simulink model "model"  (R2014a)
(part 6 of 6)

  _CN_132159930_220000_CN_132517028_220000/RConn3 -- T_132517028__Ruwais/LConn3 -- _CN_95139157_220000_CN_132517028_220000/LConn3 -- bus236/LConn1
  _CN_247122500_220000_CN_354672632_220000/LConn1 -- T_247122500__/LConn1 -- _CN_247122500_220000_CN_115677414_220000/LConn1
  _CN_247122500_220000_CN_354672632_220000/LConn2 -- T_247122500__/LConn2 -- _CN_247122500_220000_CN_115677414_220000/LConn2
  _CN_247122500_220000_CN_354672632_220000/LConn3 -- T_247122500__/LConn3 -- _CN_247122500_220000_CN_115677414_220000/LConn3 -- bus237/LConn1
  _CN_247122500_220000_CN_354672632_220000/RConn1 -- T_354672632__/LConn1 -- _CN_60234385_220000_CN_354672632_220000/LConn1 -- _CN_115677414_220000_CN_354672632_220000/LConn1
  _CN_247122500_220000_CN_354672632_220000/RConn2 -- T_354672632__/LConn2 -- _CN_60234385_220000_CN_354672632_220000/LConn2 -- _CN_115677414_220000_CN_354672632_220000/LConn2
  _CN_247122500_220000_CN_354672632_220000/RConn3 -- T_354672632__/LConn3 -- _CN_60234385_220000_CN_354672632_220000/LConn3 -- bus238/LConn1 -- _CN_115677414_220000_CN_354672632_220000/LConn3
  _CN_247122500_220000_CN_115677414_220000/RConn1 -- T_115677414__/LConn1 -- _CN_354672631_220000_CN_115677414_220000/RConn1 -- _CN_115677398_220000_CN_115677414_220000/LConn1 -- _CN_115677414_220000_CN_386199541_220000/LConn1 -- _CN_115677414_220000_CN_354672632_220000/RConn1
  _CN_247122500_220000_CN_115677414_220000/RConn2 -- T_115677414__/LConn2 -- _CN_354672631_220000_CN_115677414_220000/RConn2 -- _CN_115677398_220000_CN_115677414_220000/LConn2 -- _CN_115677414_220000_CN_386199541_220000/LConn2 -- _CN_115677414_220000_CN_354672632_220000/RConn2
  _CN_247122500_220000_CN_115677414_220000/RConn3 -- T_115677414__/LConn3 -- _CN_354672631_220000_CN_115677414_220000/RConn3 -- _CN_115677398_220000_CN_115677414_220000/LConn3 -- _CN_115677414_220000_CN_386199541_220000/LConn3 -- _CN_115677414_220000_CN_354672632_220000/RConn3 -- bus239/LConn1
  T_95099973__Liwa/LConn1 -- _CN_95099973_220000_CN_95099964_220000/RConn1
  T_95099973__Liwa/LConn2 -- _CN_95099973_220000_CN_95099964_220000/RConn2
  _CN_95099973_220000_CN_95099964_220000/RConn3 -- T_95099973__Liwa/LConn3 -- bus240/LConn1
  _CN_95139157_220000_CN_132517028_220000/RConn1 -- T_95139157__Shuweihat/RConn1 -- L_95139157/LConn1
  _CN_95139157_220000_CN_132517028_220000/RConn2 -- T_95139157__Shuweihat/RConn2 -- L_95139157/LConn2
  _CN_95139157_220000_CN_132517028_220000/RConn3 -- T_95139157__Shuweihat/RConn3 -- L_95139157/LConn3 -- bus241/LConn1
  _CN_115677398_220000_CN_115677409_220000/LConn1 -- T_115677398__/LConn1 -- _CN_115677398_220000_CN_386199534_220000/LConn1 -- _CN_115677398_220000_CN_115677414_220000/RConn1 -- _CN_115677398_220000_CN_386199505_220000/LConn1
  _CN_115677398_220000_CN_115677409_220000/LConn2 -- T_115677398__/LConn2 -- _CN_115677398_220000_CN_386199534_220000/LConn2 -- _CN_115677398_220000_CN_115677414_220000/RConn2 -- _CN_115677398_220000_CN_386199505_220000/LConn2
  _CN_115677398_220000_CN_115677409_220000/LConn3 -- T_115677398__/LConn3 -- _CN_115677398_220000_CN_386199534_220000/LConn3 -- _CN_115677398_220000_CN_115677414_220000/RConn3 -- bus242/LConn1 -- _CN_115677398_220000_CN_386199505_220000/LConn3
  G_115677409_/RConn1 -- _CN_115677398_220000_CN_115677409_220000/RConn1
  G_115677409_/RConn2 -- _CN_115677398_220000_CN_115677409_220000/RConn2
  _CN_115677398_220000_CN_115677409_220000/RConn3 -- G_115677409_/RConn3 -- bus243/LConn1
  G_386199505_/RConn1 -- _CN_115677398_220000_CN_386199505_220000/RConn1
  G_386199505_/RConn2 -- _CN_115677398_220000_CN_386199505_220000/RConn2
  _CN_115677398_220000_CN_386199505_220000/RConn3 -- G_386199505_/RConn3 -- bus244/LConn1
  _CN_115677398_220000_CN_386199534_220000/RConn1 -- T_386199534__/LConn1 -- _CN_386199534_220000_CN_386199541_220000/LConn1
  _CN_115677398_220000_CN_386199534_220000/RConn2 -- T_386199534__/LConn2 -- _CN_386199534_220000_CN_386199541_220000/LConn2
  _CN_115677398_220000_CN_386199534_220000/RConn3 -- T_386199534__/LConn3 -- _CN_386199534_220000_CN_386199541_220000/LConn3 -- bus245/LConn1
  _CN_200057688_220000_CN_95084793_220000/RConn1 -- T_95084793__/LConn1 -- _CN_95084771_220000_CN_95084793_220000/RConn1
  _CN_200057688_220000_CN_95084793_220000/RConn2 -- T_95084793__/LConn2 -- _CN_95084771_220000_CN_95084793_220000/RConn2
  _CN_200057688_220000_CN_95084793_220000/RConn3 -- T_95084793__/LConn3 -- _CN_95084771_220000_CN_95084793_220000/RConn3 -- bus246/LConn1
  _CN_115677414_220000_CN_386199541_220000/RConn1 -- T_386199541__/LConn1 -- _CN_386199534_220000_CN_386199541_220000/RConn1
  _CN_115677414_220000_CN_386199541_220000/RConn2 -- T_386199541__/LConn2 -- _CN_386199534_220000_CN_386199541_220000/RConn2
  _CN_115677414_220000_CN_386199541_220000/RConn3 -- T_386199541__/LConn3 -- _CN_386199534_220000_CN_386199541_220000/RConn3 -- bus247/LConn1
  T_60234385__/LConn1 -- _CN_60234385_220000_CN_354672632_220000/RConn1
  T_60234385__/LConn2 -- _CN_60234385_220000_CN_354672632_220000/RConn2
  _CN_60234385_220000_CN_354672632_220000/RConn3 -- T_60234385__/LConn3 -- bus248/LConn1
  _CN_95099964_220000_CN_95139199_220000/RConn1 -- T_95139199__Mirfa/RConn1 -- L_95139199/LConn1
  _CN_95099964_220000_CN_95139199_220000/RConn2 -- T_95139199__Mirfa/RConn2 -- L_95139199/LConn2
  _CN_95099964_220000_CN_95139199_220000/RConn3 -- T_95139199__Mirfa/RConn3 -- L_95139199/LConn3 -- bus249/LConn1
  T_198365955__/LConn1 -- _CN_198365955_230000_CN_199091189_230000/LConn1
  T_198365955__/LConn2 -- _CN_198365955_230000_CN_199091189_230000/LConn2
  _CN_198365955_230000_CN_199091189_230000/LConn3 -- T_198365955__/LConn3 -- bus250/LConn1
  T_199091189__/LConn1 -- _CN_198365955_230000_CN_199091189_230000/RConn1
  T_199091189__/LConn2 -- _CN_198365955_230000_CN_199091189_230000/RConn2
  _CN_198365955_230000_CN_199091189_230000/RConn3 -- T_199091189__/LConn3 -- bus251/LConn1
  T_46971910__/LConn1 -- _CN_46971910_230000_CN_197436611_230000/LConn1
  T_46971910__/LConn2 -- _CN_46971910_230000_CN_197436611_230000/LConn2
  _CN_46971910_230000_CN_197436611_230000/LConn3 -- T_46971910__/LConn3 -- bus252/LConn1
  _CN_46971910_230000_CN_197436611_230000/RConn1 -- G_197436611_/RConn1 -- _CN_197445313_230000_CN_197436611_230000/LConn1 -- _CN_132976488_230000_CN_197436611_230000/LConn1 -- _CN_197662314_230000_CN_197436611_230000/LConn1 -- _CN_197432428_230000_CN_197436611_230000/LConn1 -- _CN_132978605_380000_CN_197436611_230000/LConn1 -- _CN_197252542_380000_CN_197436611_230000/LConn1
  _CN_46971910_230000_CN_197436611_230000/RConn2 -- G_197436611_/RConn2 -- _CN_197445313_230000_CN_197436611_230000/LConn2 -- _CN_132976488_230000_CN_197436611_230000/LConn2 -- _CN_197662314_230000_CN_197436611_230000/LConn2 -- _CN_197432428_230000_CN_197436611_230000/LConn2 -- _CN_132978605_380000_CN_197436611_230000/LConn2 -- _CN_197252542_380000_CN_197436611_230000/LConn2
  _CN_46971910_230000_CN_197436611_230000/RConn3 -- G_197436611_/RConn3 -- _CN_197445313_230000_CN_197436611_230000/LConn3 -- _CN_132976488_230000_CN_197436611_230000/LConn3 -- _CN_197662314_230000_CN_197436611_230000/LConn3 -- _CN_197432428_230000_CN_197436611_230000/LConn3 -- _CN_132978605_380000_CN_197436611_230000/LConn3 -- _CN_197252542_380000_CN_197436611_230000/LConn3 -- bus253/LConn1
  _CN_198351119_230000_CN_198331310_230000/LConn1 -- T_198351119__/LConn1 -- _CN_198351119_230000_CN_198330048_230000/LConn1 -- _CN_198351119_230000_CN_132978605_230000/LConn1 -- _CN_198351119_230000_CN_132976488_230000/LConn1 -- _CN_198351119_230000_CN_198342216_230000/LConn1
  _CN_198351119_230000_CN_198331310_230000/LConn2 -- T_198351119__/LConn2 -- _CN_198351119_230000_CN_198330048_230000/LConn2 -- _CN_198351119_230000_CN_132978605_230000/LConn2 -- _CN_198351119_230000_CN_132976488_230000/LConn2 -- _CN_198351119_230000_CN_198342216_230000/LConn2
  _CN_198351119_230000_CN_198331310_230000/LConn3 -- T_198351119__/LConn3 -- _CN_198351119_230000_CN_198330048_230000/LConn3 -- _CN_198351119_230000_CN_132978605_230000/LConn3 -- _CN_198351119_230000_CN_132976488_230000/LConn3 -- _CN_198351119_230000_CN_198342216_230000/LConn3 -- bus254/LConn1
  _CN_198351119_230000_CN_198331310_230000/RConn1 -- T_198331310__/LConn1 -- _CN_198334634_230000_CN_198331310_230000/LConn1 -- _CN_132978605_230000_CN_198331310_230000/LConn1
  _CN_198351119_230000_CN_198331310_230000/RConn2 -- T_198331310__/LConn2 -- _CN_198334634_230000_CN_198331310_230000/LConn2 -- _CN_132978605_230000_CN_198331310_230000/LConn2
  _CN_198351119_230000_CN_198331310_230000/RConn3 -- T_198331310__/LConn3 -- _CN_198334634_230000_CN_198331310_230000/LConn3 -- _CN_132978605_230000_CN_198331310_230000/LConn3 -- bus255/LConn1
  T_198330048__/LConn1 -- _CN_198351119_230000_CN_198330048_230000/RConn1
  T_198330048__/LConn2 -- _CN_198351119_230000_CN_198330048_230000/RConn2
  _CN_198351119_230000_CN_198330048_230000/RConn3 -- T_198330048__/LConn3 -- bus256/LConn1
  _CN_198351119_230000_CN_132978605_230000/RConn1 -- T_132978605__/RConn1 -- _CN_132978605_230000_CN_198144511_230000/LConn1 -- _CN_132978605_230000_CN_198331310_230000/RConn1 -- L_132978605/LConn1
  _CN_198351119_230000_CN_132978605_230000/RConn2 -- T_132978605__/RConn2 -- _CN_132978605_230000_CN_198144511_230000/LConn2 -- _CN_132978605_230000_CN_198331310_230000/RConn2 -- L_132978605/LConn2
  _CN_198351119_230000_CN_132978605_230000/RConn3 -- T_132978605__/RConn3 -- _CN_132978605_230000_CN_198144511_230000/LConn3 -- _CN_132978605_230000_CN_198331310_230000/RConn3 -- L_132978605/LConn3 -- bus257/LConn1
  _CN_198351119_230000_CN_132976488_230000/RConn1 -- T_132976488__Berri_Gas_Plant/LConn1 -- _CN_132976488_230000_CN_197436611_230000/RConn1 -- _CN_132976488_230000_CN_198144511_230000/LConn1
  _CN_198351119_230000_CN_132976488_230000/RConn2 -- T_132976488__Berri_Gas_Plant/LConn2 -- _CN_132976488_230000_CN_197436611_230000/RConn2 -- _CN_132976488_230000_CN_198144511_230000/LConn2
  _CN_198351119_230000_CN_132976488_230000/RConn3 -- T_132976488__Berri_Gas_Plant/LConn3 -- _CN_132976488_230000_CN_197436611_230000/RConn3 -- bus258/LConn1 -- _CN_132976488_230000_CN_198144511_230000/LConn3
  T_198342216__/LConn1 -- _CN_198351119_230000_CN_198342216_230000/RConn1
  T_198342216__/LConn2 -- _CN_198351119_230000_CN_198342216_230000/RConn2
  _CN_198351119_230000_CN_198342216_230000/RConn3 -- T_198342216__/LConn3 -- bus259/LConn1
  _CN_168652821_230000_CN_198358326_230000/LConn1 -- T_168652821__/LConn1 -- _CN_168652821_230000_CN_188546296_230000/LConn1
  _CN_168652821_230000_CN_198358326_230000/LConn2 -- T_168652821__/LConn2 -- _CN_168652821_230000_CN_188546296_230000/LConn2
  _CN_168652821_230000_CN_198358326_230000/LConn3 -- T_168652821__/LConn3 -- _CN_168652821_230000_CN_188546296_230000/LConn3 -- bus260/LConn1
  T_198358326__/LConn1 -- _CN_168652821_230000_CN_198358326_230000/RConn1
  T_198358326__/LConn2 -- _CN_168652821_230000_CN_198358326_230000/RConn2
  _CN_168652821_230000_CN_198358326_230000/RConn3 -- T_198358326__/LConn3 -- bus261/LConn1
  T_188546296__/LConn1 -- _CN_168652821_230000_CN_188546296_230000/RConn1
  T_188546296__/LConn2 -- _CN_168652821_230000_CN_188546296_230000/RConn2
  _CN_168652821_230000_CN_188546296_230000/RConn3 -- T_188546296__/LConn3 -- bus262/LConn1
  T_198334634__/LConn1 -- _CN_198334634_230000_CN_198331310_230000/RConn1
  T_198334634__/LConn2 -- _CN_198334634_230000_CN_198331310_230000/RConn2
  _CN_198334634_230000_CN_198331310_230000/RConn3 -- T_198334634__/LConn3 -- bus263/LConn1
  _CN_132978605_230000_CN_198144511_230000/RConn1 -- T_198144511__/LConn1 -- _CN_197662314_230000_CN_198144511_230000/LConn1 -- _CN_132976488_230000_CN_198144511_230000/RConn1
  _CN_132978605_230000_CN_198144511_230000/RConn2 -- T_198144511__/LConn2 -- _CN_197662314_230000_CN_198144511_230000/LConn2 -- _CN_132976488_230000_CN_198144511_230000/RConn2
  _CN_132978605_230000_CN_198144511_230000/RConn3 -- T_198144511__/LConn3 -- _CN_197662314_230000_CN_198144511_230000/LConn3 -- bus264/LConn1 -- _CN_132976488_230000_CN_198144511_230000/RConn3
  T_195637944__/LConn1 -- _CN_195637944_230000_CN_115326815_230000/LConn1
  T_195637944__/LConn2 -- _CN_195637944_230000_CN_115326815_230000/LConn2
  _CN_195637944_230000_CN_115326815_230000/LConn3 -- T_195637944__/LConn3 -- bus265/LConn1
  _CN_195637944_230000_CN_115326815_230000/RConn1 -- T_115326815_380000_/RConn1 -- _CN_115326815_230000_CN_115326819_230000/LConn1 -- L_115326815/LConn1 -- _CN_168648926_230000_CN_115326815_230000/LConn1
  _CN_195637944_230000_CN_115326815_230000/RConn2 -- T_115326815_380000_/RConn2 -- _CN_115326815_230000_CN_115326819_230000/LConn2 -- L_115326815/LConn2 -- _CN_168648926_230000_CN_115326815_230000/LConn2
  _CN_195637944_230000_CN_115326815_230000/RConn3 -- T_115326815_380000_/RConn3 -- _CN_115326815_230000_CN_115326819_230000/LConn3 -- L_115326815/LConn3 -- bus266/LConn1 -- _CN_168648926_230000_CN_115326815_230000/LConn3
  T_197445313__/LConn1 -- _CN_197445313_230000_CN_197436611_230000/RConn1
  T_197445313__/LConn2 -- _CN_197445313_230000_CN_197436611_230000/RConn2
  _CN_197445313_230000_CN_197436611_230000/RConn3 -- T_197445313__/LConn3 -- bus267/LConn1
  T_168648926__/LConn1 -- _CN_168648926_230000_CN_115326815_230000/RConn1
  T_168648926__/LConn2 -- _CN_168648926_230000_CN_115326815_230000/RConn2
  _CN_168648926_230000_CN_115326815_230000/RConn3 -- T_168648926__/LConn3 -- bus268/LConn1
  T_115326819__/LConn1 -- _CN_115326815_230000_CN_115326819_230000/RConn1
  T_115326819__/LConn2 -- _CN_115326815_230000_CN_115326819_230000/RConn2
  _CN_115326815_230000_CN_115326819_230000/RConn3 -- T_115326819__/LConn3 -- bus269/LConn1
  _CN_197662314_230000_CN_198144511_230000/RConn1 -- T_197662314__/LConn1 -- _CN_197662314_230000_CN_197436611_230000/RConn1
  _CN_197662314_230000_CN_198144511_230000/RConn2 -- T_197662314__/LConn2 -- _CN_197662314_230000_CN_197436611_230000/RConn2
  _CN_197662314_230000_CN_198144511_230000/RConn3 -- T_197662314__/LConn3 -- _CN_197662314_230000_CN_197436611_230000/RConn3 -- bus270/LConn1
  _CN_197432428_230000_CN_197442799_230000/LConn1 -- T_197432428__/LConn1 -- _CN_197432428_230000_CN_197439486_230000/LConn1 -- _CN_197432428_230000_CN_197436611_230000/RConn1
  _CN_197432428_230000_CN_197442799_230000/LConn2 -- T_197432428__/LConn2 -- _CN_197432428_230000_CN_197439486_230000/LConn2 -- _CN_197432428_230000_CN_197436611_230000/RConn2
  _CN_197432428_230000_CN_197442799_230000/LConn3 -- T_197432428__/LConn3 -- _CN_197432428_230000_CN_197439486_230000/LConn3 -- bus271/LConn1 -- _CN_197432428_230000_CN_197436611_230000/RConn3
  T_197442799__/LConn1 -- _CN_197432428_230000_CN_197442799_230000/RConn1
  T_197442799__/LConn2 -- _CN_197432428_230000_CN_197442799_230000/RConn2
  _CN_197432428_230000_CN_197442799_230000/RConn3 -- T_197442799__/LConn3 -- bus272/LConn1
  T_197439486__/LConn1 -- _CN_197432428_230000_CN_197439486_230000/RConn1
  T_197439486__/LConn2 -- _CN_197432428_230000_CN_197439486_230000/RConn2
  _CN_197432428_230000_CN_197439486_230000/RConn3 -- T_197439486__/LConn3 -- bus273/LConn1
  T_261938325__/LConn1 -- _CN_261938325_275000_CN_160398714_275000/LConn1
  T_261938325__/LConn2 -- _CN_261938325_275000_CN_160398714_275000/LConn2
  _CN_261938325_275000_CN_160398714_275000/LConn3 -- T_261938325__/LConn3 -- bus274/LConn1
  _CN_261938325_275000_CN_160398714_275000/RConn1 -- T_160398714__/LConn1 -- _CN_261938316_275000_CN_160398714_275000/LConn1
  _CN_261938325_275000_CN_160398714_275000/RConn2 -- T_160398714__/LConn2 -- _CN_261938316_275000_CN_160398714_275000/LConn2
  _CN_261938325_275000_CN_160398714_275000/RConn3 -- T_160398714__/LConn3 -- _CN_261938316_275000_CN_160398714_275000/LConn3 -- bus275/LConn1
  T_203618603__/LConn1 -- _CN_203618603_275000_CN_132154027_275000/LConn1
  T_203618603__/LConn2 -- _CN_203618603_275000_CN_132154027_275000/LConn2
  _CN_203618603_275000_CN_132154027_275000/LConn3 -- T_203618603__/LConn3 -- bus276/LConn1
  _CN_203618603_275000_CN_132154027_275000/RConn1 -- T_132154027__/LConn1 -- _CN_203622086_275000_CN_132154027_275000/LConn1 -- _CN_132154027_275000_CN_204277162_275000/LConn1 -- _CN_132154027_275000_CN_203855651_275000/LConn1 -- _CN_132154027_275000_CN_132889809_275000/LConn1 -- _CN_132154027_275000_CN_132154028_275000/LConn1
  _CN_203618603_275000_CN_132154027_275000/RConn2 -- T_132154027__/LConn2 -- _CN_203622086_275000_CN_132154027_275000/LConn2 -- _CN_132154027_275000_CN_204277162_275000/LConn2 -- _CN_132154027_275000_CN_203855651_275000/LConn2 -- _CN_132154027_275000_CN_132889809_275000/LConn2 -- _CN_132154027_275000_CN_132154028_275000/LConn2
  _CN_203618603_275000_CN_132154027_275000/RConn3 -- T_132154027__/LConn3 -- _CN_203622086_275000_CN_132154027_275000/LConn3 -- _CN_132154027_275000_CN_204277162_275000/LConn3 -- _CN_132154027_275000_CN_203855651_275000/LConn3 -- _CN_132154027_275000_CN_132889809_275000/LConn3 -- _CN_132154027_275000_CN_132154028_275000/LConn3 -- bus277/LConn1
  T_203622084__/LConn1 -- _CN_203622084_275000_CN_204277162_275000/LConn1
  T_203622084__/LConn2 -- _CN_203622084_275000_CN_204277162_275000/LConn2
  _CN_203622084_275000_CN_204277162_275000/LConn3 -- T_203622084__/LConn3 -- bus278/LConn1
  _CN_203622084_275000_CN_204277162_275000/RConn1 -- G_204277162_Al_Zour_Thermal_Power_Plant/RConn1 -- _CN_132154027_275000_CN_204277162_275000/RConn1 -- _CN_204276494_275000_CN_204277162_275000/LConn1 -- _CN_203618746_275000_CN_204277162_275000/LConn1
  _CN_203622084_275000_CN_204277162_275000/RConn2 -- G_204277162_Al_Zour_Thermal_Power_Plant/RConn2 -- _CN_132154027_275000_CN_204277162_275000/RConn2 -- _CN_204276494_275000_CN_204277162_275000/LConn2 -- _CN_203618746_275000_CN_204277162_275000/LConn2
  _CN_203622084_275000_CN_204277162_275000/RConn3 -- G_204277162_Al_Zour_Thermal_Power_Plant/RConn3 -- _CN_132154027_275000_CN_204277162_275000/RConn3 -- _CN_204276494_275000_CN_204277162_275000/LConn3 -- _CN_203618746_275000_CN_204277162_275000/LConn3 -- bus279/LConn1
  T_203622086__/LConn1 -- _CN_203622086_275000_CN_132154027_275000/RConn1
  T_203622086__/LConn2 -- _CN_203622086_275000_CN_132154027_275000/RConn2
  _CN_203622086_275000_CN_132154027_275000/RConn3 -- T_203622086__/LConn3 -- bus280/LConn1
  T_203622279__/LConn1 -- _CN_203622279_275000_CN_132889809_275000/LConn1
  T_203622279__/LConn2 -- _CN_203622279_275000_CN_132889809_275000/LConn2
  _CN_203622279_275000_CN_132889809_275000/LConn3 -- T_203622279__/LConn3 -- bus281/LConn1
  _CN_203622279_275000_CN_132889809_275000/RConn1 -- T_132889809__/LConn1 -- _CN_132154027_275000_CN_132889809_275000/RConn1 -- _CN_203858094_275000_CN_132889809_275000/LConn1
  _CN_203622279_275000_CN_132889809_275000/RConn2 -- T_132889809__/LConn2 -- _CN_132154027_275000_CN_132889809_275000/RConn2 -- _CN_203858094_275000_CN_132889809_275000/LConn2
  _CN_203622279_275000_CN_132889809_275000/RConn3 -- T_132889809__/LConn3 -- _CN_132154027_275000_CN_132889809_275000/RConn3 -- _CN_203858094_275000_CN_132889809_275000/LConn3 -- bus282/LConn1
  "T_261938316__Substation_Al_Omariya_\"W\""/LConn1 -- _CN_261938316_275000_CN_160398714_275000/RConn1
  "T_261938316__Substation_Al_Omariya_\"W\""/LConn2 -- _CN_261938316_275000_CN_160398714_275000/RConn2
  _CN_261938316_275000_CN_160398714_275000/RConn3 -- "T_261938316__Substation_Al_Omariya_\"W\""/LConn3 -- bus283/LConn1
  _CN_132154027_275000_CN_203855651_275000/RConn1 -- T_203855651__/LConn1 -- _CN_132154028_275000_CN_203855651_275000/LConn1
  _CN_132154027_275000_CN_203855651_275000/RConn2 -- T_203855651__/LConn2 -- _CN_132154028_275000_CN_203855651_275000/LConn2
  _CN_132154027_275000_CN_203855651_275000/RConn3 -- T_203855651__/LConn3 -- _CN_132154028_275000_CN_203855651_275000/LConn3 -- bus284/LConn1
  _CN_132154027_275000_CN_132154028_275000/RConn1 -- T_132154028__Substation/LConn1 -- _CN_132154028_275000_CN_203855651_275000/RConn1
  _CN_132154027_275000_CN_132154028_275000/RConn2 -- T_132154028__Substation/LConn2 -- _CN_132154028_275000_CN_203855651_275000/RConn2
  _CN_132154027_275000_CN_132154028_275000/RConn3 -- T_132154028__Substation/LConn3 -- _CN_132154028_275000_CN_203855651_275000/RConn3 -- bus285/LConn1
  T_203858094__/LConn1 -- _CN_203858094_275000_CN_132889809_275000/RConn1
  T_203858094__/LConn2 -- _CN_203858094_275000_CN_132889809_275000/RConn2
  _CN_203858094_275000_CN_132889809_275000/RConn3 -- T_203858094__/LConn3 -- bus286/LConn1
  _CN_204276494_275000_CN_204277162_275000/RConn1 -- T_204276494__/RConn1 -- L_204276494/LConn1
  _CN_204276494_275000_CN_204277162_275000/RConn2 -- T_204276494__/RConn2 -- L_204276494/LConn2
  _CN_204276494_275000_CN_204277162_275000/RConn3 -- T_204276494__/RConn3 -- L_204276494/LConn3 -- bus287/LConn1
  T_203618746__/LConn1 -- _CN_203618746_275000_CN_204277162_275000/RConn1
  T_203618746__/LConn2 -- _CN_203618746_275000_CN_204277162_275000/RConn2
  _CN_203618746_275000_CN_204277162_275000/RConn3 -- T_203618746__/LConn3 -- bus288/LConn1
  _CN_196903043_380000_CN_115345577_380000/LConn1 -- T_196903043__/LConn1 -- _CN_196903043_380000_CN_115326815_380000/LConn1 -- _CN_196903043_380000_CN_196917881_380000/LConn1
  _CN_196903043_380000_CN_115345577_380000/LConn2 -- T_196903043__/LConn2 -- _CN_196903043_380000_CN_115326815_380000/LConn2 -- _CN_196903043_380000_CN_196917881_380000/LConn2
  _CN_196903043_380000_CN_115345577_380000/LConn3 -- T_196903043__/LConn3 -- _CN_196903043_380000_CN_115326815_380000/LConn3 -- _CN_196903043_380000_CN_196917881_380000/LConn3 -- bus289/LConn1
  _CN_196903043_380000_CN_115345577_380000/RConn1 -- T_115345577__/LConn1 -- _CN_115345577_380000_CN_195636040_380000/LConn1 -- _CN_115345577_380000_CN_115326815_380000/LConn1
  _CN_196903043_380000_CN_115345577_380000/RConn2 -- T_115345577__/LConn2 -- _CN_115345577_380000_CN_195636040_380000/LConn2 -- _CN_115345577_380000_CN_115326815_380000/LConn2
  _CN_196903043_380000_CN_115345577_380000/RConn3 -- T_115345577__/LConn3 -- _CN_115345577_380000_CN_195636040_380000/LConn3 -- _CN_115345577_380000_CN_115326815_380000/LConn3 -- bus290/LConn1
  _CN_196903043_380000_CN_115326815_380000/RConn1 -- T_115326815_380000_/LConn1 -- _CN_115326815_380000_CN_196291944_380000/LConn1 -- _CN_115345577_380000_CN_115326815_380000/RConn1
  _CN_196903043_380000_CN_115326815_380000/RConn2 -- T_115326815_380000_/LConn2 -- _CN_115326815_380000_CN_196291944_380000/LConn2 -- _CN_115345577_380000_CN_115326815_380000/RConn2
  _CN_196903043_380000_CN_115326815_380000/RConn3 -- T_115326815_380000_/LConn3 -- _CN_115326815_380000_CN_196291944_380000/LConn3 -- bus291/LConn1 -- _CN_115345577_380000_CN_115326815_380000/RConn3
  _CN_196903043_380000_CN_196917881_380000/RConn1 -- T_196917881__/LConn1 -- _CN_197434236_380000_CN_196917881_380000/LConn1
  _CN_196903043_380000_CN_196917881_380000/RConn2 -- T_196917881__/LConn2 -- _CN_197434236_380000_CN_196917881_380000/LConn2
  _CN_196903043_380000_CN_196917881_380000/RConn3 -- T_196917881__/LConn3 -- _CN_197434236_380000_CN_196917881_380000/LConn3 -- bus292/LConn1
  _CN_187924742_380000_CN_195155645_380000/LConn1 -- T_187924742__/LConn1 -- _CN_187924742_380000_CN_121847629_380000/LConn1 -- _CN_187924742_380000_CN_181132741_380000/LConn1
  _CN_187924742_380000_CN_195155645_380000/LConn2 -- T_187924742__/LConn2 -- _CN_187924742_380000_CN_121847629_380000/LConn2 -- _CN_187924742_380000_CN_181132741_380000/LConn2
  _CN_187924742_380000_CN_195155645_380000/LConn3 -- T_187924742__/LConn3 -- _CN_187924742_380000_CN_121847629_380000/LConn3 -- _CN_187924742_380000_CN_181132741_380000/LConn3 -- bus293/LConn1
  _CN_187924742_380000_CN_195155645_380000/RConn1 -- G_195155645_/RConn1 -- _CN_115345550_380000_CN_195155645_380000/LConn1 -- _CN_195156716_380000_CN_195155645_380000/LConn1
  _CN_187924742_380000_CN_195155645_380000/RConn2 -- G_195155645_/RConn2 -- _CN_115345550_380000_CN_195155645_380000/LConn2 -- _CN_195156716_380000_CN_195155645_380000/LConn2
  _CN_187924742_380000_CN_195155645_380000/RConn3 -- G_195155645_/RConn3 -- _CN_115345550_380000_CN_195155645_380000/LConn3 -- _CN_195156716_380000_CN_195155645_380000/LConn3 -- bus294/LConn1
  _CN_187924742_380000_CN_121847629_380000/RConn1 -- T_121847629__/LConn1 -- _CN_168652806_380000_CN_121847629_380000/LConn1 -- _CN_190221971_380000_CN_121847629_380000/LConn1
  _CN_187924742_380000_CN_121847629_380000/RConn2 -- T_121847629__/LConn2 -- _CN_168652806_380000_CN_121847629_380000/LConn2 -- _CN_190221971_380000_CN_121847629_380000/LConn2
  _CN_187924742_380000_CN_121847629_380000/RConn3 -- T_121847629__/LConn3 -- _CN_168652806_380000_CN_121847629_380000/LConn3 -- bus295/LConn1 -- _CN_190221971_380000_CN_121847629_380000/LConn3
  T_181132741__/LConn1 -- _CN_187924742_380000_CN_181132741_380000/RConn1
  T_181132741__/LConn2 -- _CN_187924742_380000_CN_181132741_380000/RConn2
  _CN_187924742_380000_CN_181132741_380000/RConn3 -- T_181132741__/LConn3 -- bus296/LConn1
  _CN_331253129_380000_CN_115345561_380000/LConn1 -- T_331253129__/LConn1 -- _CN_331253129_380000_CN_168652806_380000/LConn1
  _CN_331253129_380000_CN_115345561_380000/LConn2 -- T_331253129__/LConn2 -- _CN_331253129_380000_CN_168652806_380000/LConn2
  _CN_331253129_380000_CN_115345561_380000/LConn3 -- T_331253129__/LConn3 -- _CN_331253129_380000_CN_168652806_380000/LConn3 -- bus297/LConn1
  _CN_331253129_380000_CN_115345561_380000/RConn1 -- T_115345561__/LConn1 -- _CN_115345561_380000_CN_195636040_380000/LConn1
  _CN_331253129_380000_CN_115345561_380000/RConn2 -- T_115345561__/LConn2 -- _CN_115345561_380000_CN_195636040_380000/LConn2
  _CN_331253129_380000_CN_115345561_380000/RConn3 -- T_115345561__/LConn3 -- _CN_115345561_380000_CN_195636040_380000/LConn3 -- bus298/LConn1
  _CN_331253129_380000_CN_168652806_380000/RConn1 -- T_168652806__/LConn1 -- _CN_168652806_380000_CN_121847629_380000/RConn1 -- _CN_132978605_380000_CN_168652806_380000/LConn1
  _CN_331253129_380000_CN_168652806_380000/RConn2 -- T_168652806__/LConn2 -- _CN_168652806_380000_CN_121847629_380000/RConn2 -- _CN_132978605_380000_CN_168652806_380000/LConn2
  _CN_331253129_380000_CN_168652806_380000/RConn3 -- T_168652806__/LConn3 -- _CN_168652806_380000_CN_121847629_380000/RConn3 -- bus299/LConn1 -- _CN_132978605_380000_CN_168652806_380000/LConn3
  _CN_115345550_380000_CN_115345535_380000/LConn1 -- T_115345550__/LConn1 -- _CN_115345550_380000_CN_195155645_380000/RConn1
  _CN_115345550_380000_CN_115345535_380000/LConn2 -- T_115345550__/LConn2 -- _CN_115345550_380000_CN_195155645_380000/RConn2
  _CN_115345550_380000_CN_115345535_380000/LConn3 -- T_115345550__/LConn3 -- _CN_115345550_380000_CN_195155645_380000/RConn3 -- bus300/LConn1
  T_115345535__/LConn1 -- _CN_115345550_380000_CN_115345535_380000/RConn1
  T_115345535__/LConn2 -- _CN_115345550_380000_CN_115345535_380000/RConn2
  _CN_115345550_380000_CN_115345535_380000/RConn3 -- T_115345535__/LConn3 -- bus301/LConn1
  T_190221971__/LConn1 -- _CN_190221971_380000_CN_121847629_380000/RConn1
  T_190221971__/LConn2 -- _CN_190221971_380000_CN_121847629_380000/RConn2
  _CN_190221971_380000_CN_121847629_380000/RConn3 -- T_190221971__/LConn3 -- bus302/LConn1
  _CN_115345561_380000_CN_195636040_380000/RConn1 -- T_195636040__/LConn1 -- _CN_115345577_380000_CN_195636040_380000/RConn1
  _CN_115345561_380000_CN_195636040_380000/RConn2 -- T_195636040__/LConn2 -- _CN_115345577_380000_CN_195636040_380000/RConn2
  _CN_115345561_380000_CN_195636040_380000/RConn3 -- T_195636040__/LConn3 -- _CN_115345577_380000_CN_195636040_380000/RConn3 -- bus303/LConn1
  T_204824991__/LConn1 -- _CN_204824991_380000_CN_194977916_380000/LConn1
  T_204824991__/LConn2 -- _CN_204824991_380000_CN_194977916_380000/LConn2
  _CN_204824991_380000_CN_194977916_380000/LConn3 -- T_204824991__/LConn3 -- bus304/LConn1
  _CN_204824991_380000_CN_194977916_380000/RConn1 -- T_194977916__/LConn1 -- _CN_194977895_380000_CN_194977916_380000/LConn1 -- _CN_204787949_380000_CN_194977916_380000/LConn1
  _CN_204824991_380000_CN_194977916_380000/RConn2 -- T_194977916__/LConn2 -- _CN_194977895_380000_CN_194977916_380000/LConn2 -- _CN_204787949_380000_CN_194977916_380000/LConn2
  _CN_204824991_380000_CN_194977916_380000/RConn3 -- T_194977916__/LConn3 -- _CN_194977895_380000_CN_194977916_380000/LConn3 -- _CN_204787949_380000_CN_194977916_380000/LConn3 -- bus305/LConn1
  T_115345572__/LConn1 -- _CN_115345572_380000_CN_115345575_380000/LConn1
  T_115345572__/LConn2 -- _CN_115345572_380000_CN_115345575_380000/LConn2
  _CN_115345572_380000_CN_115345575_380000/LConn3 -- T_115345572__/LConn3 -- bus306/LConn1
  T_115345575__/LConn1 -- _CN_115345572_380000_CN_115345575_380000/RConn1
  T_115345575__/LConn2 -- _CN_115345572_380000_CN_115345575_380000/RConn2
  _CN_115345572_380000_CN_115345575_380000/RConn3 -- T_115345575__/LConn3 -- bus307/LConn1
  T_115204773__/LConn1 -- _CN_115204773_380000_CN_203627872_380000/LConn1
  T_115204773__/LConn2 -- _CN_115204773_380000_CN_203627872_380000/LConn2
  _CN_115204773_380000_CN_203627872_380000/LConn3 -- T_115204773__/LConn3 -- bus308/LConn1
  _CN_115204773_380000_CN_203627872_380000/RConn1 -- T_203627872__/LConn1 -- _CN_203627872_380000_CN_204787949_380000/LConn1 -- _CN_203627872_380000_CN_115168464_380000/LConn1 -- _CN_203627872_380000_CN_115188425_380000/LConn1 -- _CN_203627872_380000_CN_115168488_380000/LConn1 -- _CN_203627872_380000_CN_52609387_380000/LConn1 -- _CN_203627872_380000_CN_45103712_380000/LConn1 -- _CN_203627872_380000_CN_205485383_380000/LConn1 -- _CN_203627872_380000_CN_205485574_380000/LConn1
  _CN_115204773_380000_CN_203627872_380000/RConn2 -- T_203627872__/LConn2 -- _CN_203627872_380000_CN_204787949_380000/LConn2 -- _CN_203627872_380000_CN_115168464_380000/LConn2 -- _CN_203627872_380000_CN_115188425_380000/LConn2 -- _CN_203627872_380000_CN_115168488_380000/LConn2 -- _CN_203627872_380000_CN_52609387_380000/LConn2 -- _CN_203627872_380000_CN_45103712_380000/LConn2 -- _CN_203627872_380000_CN_205485383_380000/LConn2 -- _CN_203627872_380000_CN_205485574_380000/LConn2
  _CN_115204773_380000_CN_203627872_380000/RConn3 -- T_203627872__/LConn3 -- _CN_203627872_380000_CN_204787949_380000/LConn3 -- bus309/LConn1 -- _CN_203627872_380000_CN_115168464_380000/LConn3 -- _CN_203627872_380000_CN_115188425_380000/LConn3 -- _CN_203627872_380000_CN_115168488_380000/LConn3 -- _CN_203627872_380000_CN_52609387_380000/LConn3 -- _CN_203627872_380000_CN_45103712_380000/LConn3 -- _CN_203627872_380000_CN_205485383_380000/LConn3 -- _CN_203627872_380000_CN_205485574_380000/LConn3
  _CN_132978605_380000_CN_197436611_230000/RConn1 -- T_132978605__/LConn1 -- _CN_132978605_380000_CN_168652806_380000/RConn1
  _CN_132978605_380000_CN_197436611_230000/RConn2 -- T_132978605__/LConn2 -- _CN_132978605_380000_CN_168652806_380000/RConn2
  _CN_132978605_380000_CN_197436611_230000/RConn3 -- T_132978605__/LConn3 -- _CN_132978605_380000_CN_168652806_380000/RConn3 -- bus310/LConn1
  T_197252542__/LConn1 -- _CN_197252542_380000_CN_197436611_230000/RConn1
  T_197252542__/LConn2 -- _CN_197252542_380000_CN_197436611_230000/RConn2
  _CN_197252542_380000_CN_197436611_230000/RConn3 -- T_197252542__/LConn3 -- bus311/LConn1
  _CN_203627872_380000_CN_115168464_380000/RConn1 -- T_115168464__/LConn1 -- _CN_115168464_380000_CN_115168488_380000/LConn1 -- _CN_115168464_380000_CN_115135433_380000/LConn1
  _CN_203627872_380000_CN_115168464_380000/RConn2 -- T_115168464__/LConn2 -- _CN_115168464_380000_CN_115168488_380000/LConn2 -- _CN_115168464_380000_CN_115135433_380000/LConn2
  _CN_203627872_380000_CN_115168464_380000/RConn3 -- T_115168464__/LConn3 -- _CN_115168464_380000_CN_115168488_380000/LConn3 -- _CN_115168464_380000_CN_115135433_380000/LConn3 -- bus312/LConn1
  T_115188425__/LConn1 -- _CN_203627872_380000_CN_115188425_380000/RConn1
  T_115188425__/LConn2 -- _CN_203627872_380000_CN_115188425_380000/RConn2
  _CN_203627872_380000_CN_115188425_380000/RConn3 -- T_115188425__/LConn3 -- bus313/LConn1
  _CN_203627872_380000_CN_115168488_380000/RConn1 -- T_115168488__/LConn1 -- _CN_115168464_380000_CN_115168488_380000/RConn1
  _CN_203627872_380000_CN_115168488_380000/RConn2 -- T_115168488__/LConn2 -- _CN_115168464_380000_CN_115168488_380000/RConn2
  _CN_203627872_380000_CN_115168488_380000/RConn3 -- T_115168488__/LConn3 -- _CN_115168464_380000_CN_115168488_380000/RConn3 -- bus314/LConn1
  T_52609387__/LConn1 -- _CN_203627872_380000_CN_52609387_380000/RConn1
  T_52609387__/LConn2 -- _CN_203627872_380000_CN_52609387_380000/RConn2
  _CN_203627872_380000_CN_52609387_380000/RConn3 -- T_52609387__/LConn3 -- bus315/LConn1
  T_45103712__/LConn1 -- _CN_203627872_380000_CN_45103712_380000/RConn1
  T_45103712__/LConn2 -- _CN_203627872_380000_CN_45103712_380000/RConn2
  _CN_203627872_380000_CN_45103712_380000/RConn3 -- T_45103712__/LConn3 -- bus316/LConn1
  T_205485383__/LConn1 -- _CN_203627872_380000_CN_205485383_380000/RConn1
  T_205485383__/LConn2 -- _CN_203627872_380000_CN_205485383_380000/RConn2
  _CN_203627872_380000_CN_205485383_380000/RConn3 -- T_205485383__/LConn3 -- bus317/LConn1
  T_205485574__/LConn1 -- _CN_203627872_380000_CN_205485574_380000/RConn1
  T_205485574__/LConn2 -- _CN_203627872_380000_CN_205485574_380000/RConn2
  _CN_203627872_380000_CN_205485574_380000/RConn3 -- T_205485574__/LConn3 -- bus318/LConn1
  _CN_203627872_380000_CN_204787949_380000/RConn1 -- T_204787949__/LConn1 -- _CN_204787949_380000_CN_194977916_380000/RConn1
  _CN_203627872_380000_CN_204787949_380000/RConn2 -- T_204787949__/LConn2 -- _CN_204787949_380000_CN_194977916_380000/RConn2
  _CN_203627872_380000_CN_204787949_380000/RConn3 -- T_204787949__/LConn3 -- _CN_204787949_380000_CN_194977916_380000/RConn3 -- bus319/LConn1
  G_115135433_/RConn1 -- _CN_115168464_380000_CN_115135433_380000/RConn1
  G_115135433_/RConn2 -- _CN_115168464_380000_CN_115135433_380000/RConn2
  _CN_115168464_380000_CN_115135433_380000/RConn3 -- G_115135433_/RConn3 -- bus320/LConn1
  _CN_115326806_380000_CN_207785816_380000/LConn1 -- T_115326806_380000_/LConn1 -- _CN_115326806_380000_CN_196291944_380000/LConn1
  _CN_115326806_380000_CN_207785816_380000/LConn2 -- T_115326806_380000_/LConn2 -- _CN_115326806_380000_CN_196291944_380000/LConn2
  _CN_115326806_380000_CN_207785816_380000/LConn3 -- T_115326806_380000_/LConn3 -- _CN_115326806_380000_CN_196291944_380000/LConn3 -- bus321/LConn1
  _CN_115326806_380000_CN_207785816_380000/RConn1 -- T_207785816__/LConn1 -- _CN_207785816_380000_CN_195156716_380000/LConn1
  _CN_115326806_380000_CN_207785816_380000/RConn2 -- T_207785816__/LConn2 -- _CN_207785816_380000_CN_195156716_380000/LConn2
  _CN_115326806_380000_CN_207785816_380000/RConn3 -- T_207785816__/LConn3 -- _CN_207785816_380000_CN_195156716_380000/LConn3 -- bus322/LConn1
  _CN_115326806_380000_CN_196291944_380000/RConn1 -- T_196291944__/LConn1 -- _CN_115326815_380000_CN_196291944_380000/RConn1
  _CN_115326806_380000_CN_196291944_380000/RConn2 -- T_196291944__/LConn2 -- _CN_115326815_380000_CN_196291944_380000/RConn2
  _CN_115326806_380000_CN_196291944_380000/RConn3 -- T_196291944__/LConn3 -- _CN_115326815_380000_CN_196291944_380000/RConn3 -- bus323/LConn1
  _CN_207785816_380000_CN_195156716_380000/RConn1 -- T_195156716__/LConn1 -- _CN_195156716_380000_CN_195155645_380000/RConn1
  _CN_207785816_380000_CN_195156716_380000/RConn2 -- T_195156716__/LConn2 -- _CN_195156716_380000_CN_195155645_380000/RConn2
  _CN_207785816_380000_CN_195156716_380000/RConn3 -- T_195156716__/LConn3 -- _CN_195156716_380000_CN_195155645_380000/RConn3 -- bus324/LConn1
  T_209263045__/LConn1 -- _CN_209263045_380000_CN_208619658_132000/RConn1
  T_209263045__/LConn2 -- _CN_209263045_380000_CN_208619658_132000/RConn2
  _CN_209263045_380000_CN_208619658_132000/RConn3 -- T_209263045__/LConn3 -- bus325/LConn1
  _CN_216869978_380000_CN_135035727_380000/LConn1 -- T_216869978__/LConn1 -- _CN_216869978_380000_CN_208619658_132000/RConn1
  _CN_216869978_380000_CN_135035727_380000/LConn2 -- T_216869978__/LConn2 -- _CN_216869978_380000_CN_208619658_132000/RConn2
  _CN_216869978_380000_CN_135035727_380000/LConn3 -- T_216869978__/LConn3 -- _CN_216869978_380000_CN_208619658_132000/RConn3 -- bus326/LConn1
  G_135035727_/RConn1 -- _CN_216869978_380000_CN_135035727_380000/RConn1
  G_135035727_/RConn2 -- _CN_216869978_380000_CN_135035727_380000/RConn2
  _CN_216869978_380000_CN_135035727_380000/RConn3 -- G_135035727_/RConn3 -- bus327/LConn1
  T_231599971__/LConn1 -- _CN_231599971_380000_CN_208619658_132000/RConn1
  T_231599971__/LConn2 -- _CN_231599971_380000_CN_208619658_132000/RConn2
  _CN_231599971_380000_CN_208619658_132000/RConn3 -- T_231599971__/LConn3 -- bus328/LConn1
  T_194977895__/LConn1 -- _CN_194977895_380000_CN_194977916_380000/RConn1
  T_194977895__/LConn2 -- _CN_194977895_380000_CN_194977916_380000/RConn2
  _CN_194977895_380000_CN_194977916_380000/RConn3 -- T_194977895__/LConn3 -- bus329/LConn1
  T_197434236__/LConn1 -- _CN_197434236_380000_CN_196917881_380000/RConn1
  T_197434236__/LConn2 -- _CN_197434236_380000_CN_196917881_380000/RConn2
  _CN_197434236_380000_CN_196917881_380000/RConn3 -- T_197434236__/LConn3 -- bus330/LConn1
  _CN_309146009_400000_CN_186499524_400000/LConn1 -- T_309146009__Sila/LConn1 -- _CN_309146009_400000_CN_95139157_400000/LConn1
  _CN_309146009_400000_CN_186499524_400000/LConn2 -- T_309146009__Sila/LConn2 -- _CN_309146009_400000_CN_95139157_400000/LConn2
  _CN_309146009_400000_CN_186499524_400000/LConn3 -- T_309146009__Sila/LConn3 -- _CN_309146009_400000_CN_95139157_400000/LConn3 -- bus331/LConn1
  _CN_309146009_400000_CN_186499524_400000/RConn1 -- T_186499524__Salwa/LConn1 -- _CN_186499524_400000_CN_196917879_400000/LConn1
  _CN_309146009_400000_CN_186499524_400000/RConn2 -- T_186499524__Salwa/LConn2 -- _CN_186499524_400000_CN_196917879_400000/LConn2
  _CN_309146009_400000_CN_186499524_400000/RConn3 -- T_186499524__Salwa/LConn3 -- _CN_186499524_400000_CN_196917879_400000/LConn3 -- bus332/LConn1
  _CN_309146009_400000_CN_95139157_400000/RConn1 -- T_95139157__Shuweihat/LConn1 -- _CN_259874704_400000_CN_95139157_400000/LConn1
  _CN_309146009_400000_CN_95139157_400000/RConn2 -- T_95139157__Shuweihat/LConn2 -- _CN_259874704_400000_CN_95139157_400000/LConn2
  _CN_309146009_400000_CN_95139157_400000/RConn3 -- T_95139157__Shuweihat/LConn3 -- _CN_259874704_400000_CN_95139157_400000/LConn3 -- bus333/LConn1
  _CN_385901993_400000_CN_375827318_400000/LConn1 -- T_385901993__/LConn1 -- _CN_385901993_400000_CN_29495366_400000/LConn1 -- _CN_385901993_400000_CN_29497443_400000/LConn1 -- _CN_385901993_400000_CN_29495157_400000/LConn1 -- _CN_385901993_400000_CN_173064710_400000/LConn1 -- _CN_385901993_400000_CN_29497493_400000/LConn1 -- _CN_385901993_400000_CN_94816872_400000/LConn1 -- _CN_385901993_400000_CN_359425700_400000/LConn1 -- _CN_385901993_400000_CN_155312475_400000/LConn1
  _CN_385901993_400000_CN_375827318_400000/LConn2 -- T_385901993__/LConn2 -- _CN_385901993_400000_CN_29495366_400000/LConn2 -- _CN_385901993_400000_CN_29497443_400000/LConn2 -- _CN_385901993_400000_CN_29495157_400000/LConn2 -- _CN_385901993_400000_CN_173064710_400000/LConn2 -- _CN_385901993_400000_CN_29497493_400000/LConn2 -- _CN_385901993_400000_CN_94816872_400000/LConn2 -- _CN_385901993_400000_CN_359425700_400000/LConn2 -- _CN_385901993_400000_CN_155312475_400000/LConn2
  _CN_385901993_400000_CN_375827318_400000/LConn3 -- T_385901993__/LConn3 -- _CN_385901993_400000_CN_29495366_400000/LConn3 -- _CN_385901993_400000_CN_29497443_400000/LConn3 -- _CN_385901993_400000_CN_29495157_400000/LConn3 -- _CN_385901993_400000_CN_173064710_400000/LConn3 -- _CN_385901993_400000_CN_29497493_400000/LConn3 -- _CN_385901993_400000_CN_94816872_400000/LConn3 -- _CN_385901993_400000_CN_359425700_400000/LConn3 -- bus334/LConn1 -- _CN_385901993_400000_CN_155312475_400000/LConn3
  _CN_385901993_400000_CN_375827318_400000/RConn1 -- T_375827318__/LConn1 -- _CN_29494113_400000_CN_375827318_400000/LConn1
  _CN_385901993_400000_CN_375827318_400000/RConn2 -- T_375827318__/LConn2 -- _CN_29494113_400000_CN_375827318_400000/LConn2
  _CN_385901993_400000_CN_375827318_400000/RConn3 -- T_375827318__/LConn3 -- _CN_29494113_400000_CN_375827318_400000/LConn3 -- bus335/LConn1
  _CN_385901993_400000_CN_155312475_400000/RConn1 -- G_155312475_Power_Plant/RConn1 -- _CN_181332756_400000_CN_155312475_400000/LConn1 -- _CN_94950821_400000_CN_155312475_400000/LConn1 -- _CN_29494113_400000_CN_155312475_400000/LConn1 -- _CN_375782393_400000_CN_155312475_400000/LConn1 -- _CN_375782394_400000_CN_155312475_400000/LConn1 -- _CN_24510596_400000_CN_155312475_400000/LConn1
  _CN_385901993_400000_CN_155312475_400000/RConn2 -- G_155312475_Power_Plant/RConn2 -- _CN_181332756_400000_CN_155312475_400000/LConn2 -- _CN_94950821_400000_CN_155312475_400000/LConn2 -- _CN_29494113_400000_CN_155312475_400000/LConn2 -- _CN_375782393_400000_CN_155312475_400000/LConn2 -- _CN_375782394_400000_CN_155312475_400000/LConn2 -- _CN_24510596_400000_CN_155312475_400000/LConn2
  _CN_385901993_400000_CN_155312475_400000/RConn3 -- G_155312475_Power_Plant/RConn3 -- _CN_181332756_400000_CN_155312475_400000/LConn3 -- _CN_94950821_400000_CN_155312475_400000/LConn3 -- _CN_29494113_400000_CN_155312475_400000/LConn3 -- _CN_375782393_400000_CN_155312475_400000/LConn3 -- _CN_375782394_400000_CN_155312475_400000/LConn3 -- bus336/LConn1 -- _CN_24510596_400000_CN_155312475_400000/LConn3
  T_29495366__/LConn1 -- _CN_385901993_400000_CN_29495366_400000/RConn1
  T_29495366__/LConn2 -- _CN_385901993_400000_CN_29495366_400000/RConn2
  _CN_385901993_400000_CN_29495366_400000/RConn3 -- T_29495366__/LConn3 -- bus337/LConn1
  T_29497443__/LConn1 -- _CN_385901993_400000_CN_29497443_400000/RConn1
  T_29497443__/LConn2 -- _CN_385901993_400000_CN_29497443_400000/RConn2
  _CN_385901993_400000_CN_29497443_400000/RConn3 -- T_29497443__/LConn3 -- bus338/LConn1
  _CN_385901993_400000_CN_29495157_400000/RConn1 -- T_29495157__/LConn1 -- _CN_359425700_400000_CN_29495157_400000/LConn1
  _CN_385901993_400000_CN_29495157_400000/RConn2 -- T_29495157__/LConn2 -- _CN_359425700_400000_CN_29495157_400000/LConn2
  _CN_385901993_400000_CN_29495157_400000/RConn3 -- T_29495157__/LConn3 -- _CN_359425700_400000_CN_29495157_400000/LConn3 -- bus339/LConn1
  _CN_385901993_400000_CN_173064710_400000/RConn1 -- T_173064710__/LConn1 -- _CN_173064710_400000_CN_360069074_400000/LConn1 -- _CN_173064710_400000_CN_173064712_400000/LConn1
  _CN_385901993_400000_CN_173064710_400000/RConn2 -- T_173064710__/LConn2 -- _CN_173064710_400000_CN_360069074_400000/LConn2 -- _CN_173064710_400000_CN_173064712_400000/LConn2
  _CN_385901993_400000_CN_173064710_400000/RConn3 -- T_173064710__/LConn3 -- _CN_173064710_400000_CN_360069074_400000/LConn3 -- _CN_173064710_400000_CN_173064712_400000/LConn3 -- bus340/LConn1
  T_29497493__/LConn1 -- _CN_385901993_400000_CN_29497493_400000/RConn1
  T_29497493__/LConn2 -- _CN_385901993_400000_CN_29497493_400000/RConn2
  _CN_385901993_400000_CN_29497493_400000/RConn3 -- T_29497493__/LConn3 -- bus341/LConn1
  _CN_385901993_400000_CN_94816872_400000/RConn1 -- T_94816872__/LConn1 -- _CN_181332762_400000_CN_94816872_400000/LConn1
  _CN_385901993_400000_CN_94816872_400000/RConn2 -- T_94816872__/LConn2 -- _CN_181332762_400000_CN_94816872_400000/LConn2
  _CN_385901993_400000_CN_94816872_400000/RConn3 -- T_94816872__/LConn3 -- _CN_181332762_400000_CN_94816872_400000/LConn3 -- bus342/LConn1
  _CN_385901993_400000_CN_359425700_400000/RConn1 -- T_359425700__Barsha/LConn1 -- _CN_359425700_400000_CN_29495157_400000/RConn1
  _CN_385901993_400000_CN_359425700_400000/RConn2 -- T_359425700__Barsha/LConn2 -- _CN_359425700_400000_CN_29495157_400000/RConn2
  _CN_385901993_400000_CN_359425700_400000/RConn3 -- T_359425700__Barsha/LConn3 -- _CN_359425700_400000_CN_29495157_400000/RConn3 -- bus343/LConn1
  _CN_24510596_400000_CN_155312475_400000/RConn1 -- T_24510596__/LConn1 -- _CN_24510596_400000_CN_181332757_400000/LConn1 -- _CN_24510596_400000_CN_181332762_400000/LConn1
  _CN_24510596_400000_CN_155312475_400000/RConn2 -- T_24510596__/LConn2 -- _CN_24510596_400000_CN_181332757_400000/LConn2 -- _CN_24510596_400000_CN_181332762_400000/LConn2
  _CN_24510596_400000_CN_155312475_400000/RConn3 -- T_24510596__/LConn3 -- _CN_24510596_400000_CN_181332757_400000/LConn3 -- _CN_24510596_400000_CN_181332762_400000/LConn3 -- bus344/LConn1
  T_181332757__DEWA/LConn1 -- _CN_24510596_400000_CN_181332757_400000/RConn1
  T_181332757__DEWA/LConn2 -- _CN_24510596_400000_CN_181332757_400000/RConn2
  _CN_24510596_400000_CN_181332757_400000/RConn3 -- T_181332757__DEWA/LConn3 -- bus345/LConn1
  _CN_24510596_400000_CN_181332762_400000/RConn1 -- T_181332762__/LConn1 -- _CN_181332762_400000_CN_94816872_400000/RConn1
  _CN_24510596_400000_CN_181332762_400000/RConn2 -- T_181332762__/LConn2 -- _CN_181332762_400000_CN_94816872_400000/RConn2
  _CN_24510596_400000_CN_181332762_400000/RConn3 -- T_181332762__/LConn3 -- _CN_181332762_400000_CN_94816872_400000/RConn3 -- bus346/LConn1
  G_360069074_/RConn1 -- _CN_173064710_400000_CN_360069074_400000/RConn1
  G_360069074_/RConn2 -- _CN_173064710_400000_CN_360069074_400000/RConn2
  _CN_173064710_400000_CN_360069074_400000/RConn3 -- G_360069074_/RConn3 -- bus347/LConn1
  _CN_173064710_400000_CN_173064712_400000/RConn1 -- T_173064712__/LConn1 -- _CN_173064712_400000_CN_149865727_400000/LConn1
  _CN_173064710_400000_CN_173064712_400000/RConn2 -- T_173064712__/LConn2 -- _CN_173064712_400000_CN_149865727_400000/LConn2
  _CN_173064710_400000_CN_173064712_400000/RConn3 -- T_173064712__/LConn3 -- _CN_173064712_400000_CN_149865727_400000/LConn3 -- bus348/LConn1
  _CN_173064712_400000_CN_149865727_400000/RConn1 -- T_149865727__/LConn1 -- _CN_375782394_400000_CN_149865727_400000/LConn1
  _CN_173064712_400000_CN_149865727_400000/RConn2 -- T_149865727__/LConn2 -- _CN_375782394_400000_CN_149865727_400000/LConn2
  _CN_173064712_400000_CN_149865727_400000/RConn3 -- T_149865727__/LConn3 -- _CN_375782394_400000_CN_149865727_400000/LConn3 -- bus349/LConn1
  _CN_24394891_400000_CN_94950821_400000/LConn1 -- T_24394891__/LConn1 -- _CN_24394891_400000_CN_95084799_400000/LConn1
  _CN_24394891_400000_CN_94950821_400000/LConn2 -- T_24394891__/LConn2 -- _CN_24394891_400000_CN_95084799_400000/LConn2
  _CN_24394891_400000_CN_94950821_400000/LConn3 -- T_24394891__/LConn3 -- _CN_24394891_400000_CN_95084799_400000/LConn3 -- bus350/LConn1
  _CN_24394891_400000_CN_94950821_400000/RConn1 -- T_94950821__/LConn1 -- _CN_94950821_400000_CN_155312475_400000/RConn1 -- _CN_174871442_400000_CN_94950821_400000/LConn1
  _CN_24394891_400000_CN_94950821_400000/RConn2 -- T_94950821__/LConn2 -- _CN_94950821_400000_CN_155312475_400000/RConn2 -- _CN_174871442_400000_CN_94950821_400000/LConn2
  _CN_24394891_400000_CN_94950821_400000/RConn3 -- T_94950821__/LConn3 -- _CN_94950821_400000_CN_155312475_400000/RConn3 -- bus351/LConn1 -- _CN_174871442_400000_CN_94950821_400000/LConn3
  T_95084799__Dahma/LConn1 -- _CN_24394891_400000_CN_95084799_400000/RConn1
  T_95084799__Dahma/LConn2 -- _CN_24394891_400000_CN_95084799_400000/RConn2
  _CN_24394891_400000_CN_95084799_400000/RConn3 -- T_95084799__Dahma/LConn3 -- bus352/LConn1
  T_204276494__/LConn1 -- _CN_204276494_400000_CN_198117361_400000/LConn1
  T_204276494__/LConn2 -- _CN_204276494_400000_CN_198117361_400000/LConn2
  _CN_204276494_400000_CN_198117361_400000/LConn3 -- T_204276494__/LConn3 -- bus353/LConn1
  _CN_204276494_400000_CN_198117361_400000/RConn1 -- T_198117361__Al_Fadhili_back_to_back_HVDC_converter_station/LConn1 -- _CN_196917879_400000_CN_198117361_400000/LConn1
  _CN_204276494_400000_CN_198117361_400000/RConn2 -- T_198117361__Al_Fadhili_back_to_back_HVDC_converter_station/LConn2 -- _CN_196917879_400000_CN_198117361_400000/LConn2
  _CN_204276494_400000_CN_198117361_400000/RConn3 -- T_198117361__Al_Fadhili_back_to_back_HVDC_converter_station/LConn3 -- _CN_196917879_400000_CN_198117361_400000/LConn3 -- bus354/LConn1
  _CN_259874704_400000_CN_95139157_400000/RConn1 -- T_259874704__/LConn1 -- _CN_259874704_400000_CN_29504119_400000/LConn1 -- _CN_259874704_400000_CN_95139199_400000/LConn1
  _CN_259874704_400000_CN_95139157_400000/RConn2 -- T_259874704__/LConn2 -- _CN_259874704_400000_CN_29504119_400000/LConn2 -- _CN_259874704_400000_CN_95139199_400000/LConn2
  _CN_259874704_400000_CN_95139157_400000/RConn3 -- T_259874704__/LConn3 -- _CN_259874704_400000_CN_29504119_400000/LConn3 -- bus355/LConn1 -- _CN_259874704_400000_CN_95139199_400000/LConn3
  T_95139199__Mirfa/LConn1 -- _CN_259874704_400000_CN_95139199_400000/RConn1
  T_95139199__Mirfa/LConn2 -- _CN_259874704_400000_CN_95139199_400000/RConn2
  _CN_259874704_400000_CN_95139199_400000/RConn3 -- T_95139199__Mirfa/LConn3 -- bus356/LConn1
  _CN_259874704_400000_CN_29504119_400000/RConn1 -- T_29504119__Substation/LConn1 -- _CN_94950807_400000_CN_29504119_400000/LConn1
  _CN_259874704_400000_CN_29504119_400000/RConn2 -- T_29504119__Substation/LConn2 -- _CN_94950807_400000_CN_29504119_400000/LConn2
  _CN_259874704_400000_CN_29504119_400000/RConn3 -- T_29504119__Substation/LConn3 -- _CN_94950807_400000_CN_29504119_400000/LConn3 -- bus357/LConn1
  T_174871442__/LConn1 -- _CN_174871442_400000_CN_94950821_400000/RConn1
  T_174871442__/LConn2 -- _CN_174871442_400000_CN_94950821_400000/RConn2
  _CN_174871442_400000_CN_94950821_400000/RConn3 -- T_174871442__/LConn3 -- bus358/LConn1
  _CN_260963603_400000_CN_95046953_400000/LConn1 -- T_260963603__/LConn1 -- _CN_260963603_400000_CN_301911494_400000/LConn1
  _CN_260963603_400000_CN_95046953_400000/LConn2 -- T_260963603__/LConn2 -- _CN_260963603_400000_CN_301911494_400000/LConn2
  _CN_260963603_400000_CN_95046953_400000/LConn3 -- T_260963603__/LConn3 -- _CN_260963603_400000_CN_301911494_400000/LConn3 -- bus359/LConn1
  T_95046953__Sweihan/LConn1 -- _CN_260963603_400000_CN_95046953_400000/RConn1
  T_95046953__Sweihan/LConn2 -- _CN_260963603_400000_CN_95046953_400000/RConn2
  _CN_260963603_400000_CN_95046953_400000/RConn3 -- T_95046953__Sweihan/LConn3 -- bus360/LConn1
  _CN_260963603_400000_CN_301911494_400000/RConn1 -- T_301911494__/LConn1 -- _CN_181332756_400000_CN_301911494_400000/LConn1 -- _CN_301911494_400000_CN_94816851_400000/LConn1 -- _CN_301911494_400000_CN_260963602_400000/LConn1
  _CN_260963603_400000_CN_301911494_400000/RConn2 -- T_301911494__/LConn2 -- _CN_181332756_400000_CN_301911494_400000/LConn2 -- _CN_301911494_400000_CN_94816851_400000/LConn2 -- _CN_301911494_400000_CN_260963602_400000/LConn2
  _CN_260963603_400000_CN_301911494_400000/RConn3 -- T_301911494__/LConn3 -- _CN_181332756_400000_CN_301911494_400000/LConn3 -- _CN_301911494_400000_CN_94816851_400000/LConn3 -- _CN_301911494_400000_CN_260963602_400000/LConn3 -- bus361/LConn1
  _CN_181332756_400000_CN_301911494_400000/RConn1 -- T_181332756__/LConn1 -- _CN_181332756_400000_CN_155312475_400000/RConn1 -- _CN_181332756_400000_CN_94816851_400000/LConn1 -- _CN_181332756_400000_CN_354339381_400000/LConn1
  _CN_181332756_400000_CN_301911494_400000/RConn2 -- T_181332756__/LConn2 -- _CN_181332756_400000_CN_155312475_400000/RConn2 -- _CN_181332756_400000_CN_94816851_400000/LConn2 -- _CN_181332756_400000_CN_354339381_400000/LConn2
  _CN_181332756_400000_CN_301911494_400000/RConn3 -- T_181332756__/LConn3 -- _CN_181332756_400000_CN_155312475_400000/RConn3 -- _CN_181332756_400000_CN_94816851_400000/LConn3 -- _CN_181332756_400000_CN_354339381_400000/LConn3 -- bus362/LConn1
  _CN_181332756_400000_CN_94816851_400000/RConn1 -- T_94816851__/LConn1 -- _CN_301911494_400000_CN_94816851_400000/RConn1
  _CN_181332756_400000_CN_94816851_400000/RConn2 -- T_94816851__/LConn2 -- _CN_301911494_400000_CN_94816851_400000/RConn2
  _CN_181332756_400000_CN_94816851_400000/RConn3 -- T_94816851__/LConn3 -- _CN_301911494_400000_CN_94816851_400000/RConn3 -- bus363/LConn1
  T_354339381__/LConn1 -- _CN_181332756_400000_CN_354339381_400000/RConn1
  T_354339381__/LConn2 -- _CN_181332756_400000_CN_354339381_400000/RConn2
  _CN_181332756_400000_CN_354339381_400000/RConn3 -- T_354339381__/LConn3 -- bus364/LConn1
  T_94950807__/LConn1 -- _CN_94950807_400000_CN_29504119_400000/RConn1
  T_94950807__/LConn2 -- _CN_94950807_400000_CN_29504119_400000/RConn2
  _CN_94950807_400000_CN_29504119_400000/RConn3 -- T_94950807__/LConn3 -- bus365/LConn1
  _CN_186499524_400000_CN_196917879_400000/RConn1 -- T_196917879__/LConn1 -- _CN_169873584_400000_CN_196917879_400000/LConn1 -- _CN_196917879_400000_CN_198117361_400000/RConn1
  _CN_186499524_400000_CN_196917879_400000/RConn2 -- T_196917879__/LConn2 -- _CN_169873584_400000_CN_196917879_400000/LConn2 -- _CN_196917879_400000_CN_198117361_400000/RConn2
  _CN_186499524_400000_CN_196917879_400000/RConn3 -- T_196917879__/LConn3 -- _CN_169873584_400000_CN_196917879_400000/LConn3 -- _CN_196917879_400000_CN_198117361_400000/RConn3 -- bus366/LConn1
  T_186404765__/LConn1 -- _CN_186404765_400000_CN_186404770_400000/LConn1
  T_186404765__/LConn2 -- _CN_186404765_400000_CN_186404770_400000/LConn2
  _CN_186404765_400000_CN_186404770_400000/LConn3 -- T_186404765__/LConn3 -- bus367/LConn1
  _CN_186404765_400000_CN_186404770_400000/RConn1 -- T_186404770_400000_/LConn1 -- _CN_186488516_400000_CN_186404770_400000/LConn1
  _CN_186404765_400000_CN_186404770_400000/RConn2 -- T_186404770_400000_/LConn2 -- _CN_186488516_400000_CN_186404770_400000/LConn2
  _CN_186404765_400000_CN_186404770_400000/RConn3 -- T_186404770_400000_/LConn3 -- _CN_186488516_400000_CN_186404770_400000/LConn3 -- bus368/LConn1
  T_177998754__/LConn1 -- _CN_177998754_400000_CN_321061210_400000/LConn1
  T_177998754__/LConn2 -- _CN_177998754_400000_CN_321061210_400000/LConn2
  _CN_177998754_400000_CN_321061210_400000/LConn3 -- T_177998754__/LConn3 -- bus369/LConn1
  T_321061210__/LConn1 -- _CN_177998754_400000_CN_321061210_400000/RConn1
  T_321061210__/LConn2 -- _CN_177998754_400000_CN_321061210_400000/RConn2
  _CN_177998754_400000_CN_321061210_400000/RConn3 -- T_321061210__/LConn3 -- bus370/LConn1
  T_260963602__/LConn1 -- _CN_301911494_400000_CN_260963602_400000/RConn1
  T_260963602__/LConn2 -- _CN_301911494_400000_CN_260963602_400000/RConn2
  _CN_301911494_400000_CN_260963602_400000/RConn3 -- T_260963602__/LConn3 -- bus371/LConn1
  T_169873584__/LConn1 -- _CN_169873584_400000_CN_196917879_400000/RConn1
  T_169873584__/LConn2 -- _CN_169873584_400000_CN_196917879_400000/RConn2
  _CN_169873584_400000_CN_196917879_400000/RConn3 -- T_169873584__/LConn3 -- bus372/LConn1
  _CN_186488516_400000_CN_186488517_400000/LConn1 -- T_186488516__Um_Birka_Super/LConn1 -- _CN_186488516_400000_CN_186404770_400000/RConn1
  _CN_186488516_400000_CN_186488517_400000/LConn2 -- T_186488516__Um_Birka_Super/LConn2 -- _CN_186488516_400000_CN_186404770_400000/RConn2
  _CN_186488516_400000_CN_186488517_400000/LConn3 -- T_186488516__Um_Birka_Super/LConn3 -- _CN_186488516_400000_CN_186404770_400000/RConn3 -- bus373/LConn1
  T_186488517__/LConn1 -- _CN_186488516_400000_CN_186488517_400000/RConn1
  T_186488517__/LConn2 -- _CN_186488516_400000_CN_186488517_400000/RConn2
  _CN_186488516_400000_CN_186488517_400000/RConn3 -- T_186488517__/LConn3 -- bus374/LConn1
  _CN_29494113_400000_CN_375827318_400000/RConn1 -- T_29494113__/LConn1 -- _CN_29494113_400000_CN_155312475_400000/RConn1
  _CN_29494113_400000_CN_375827318_400000/RConn2 -- T_29494113__/LConn2 -- _CN_29494113_400000_CN_155312475_400000/RConn2
  _CN_29494113_400000_CN_375827318_400000/RConn3 -- T_29494113__/LConn3 -- _CN_29494113_400000_CN_155312475_400000/RConn3 -- bus375/LConn1
  T_375782393__/LConn1 -- _CN_375782393_400000_CN_155312475_400000/RConn1
  T_375782393__/LConn2 -- _CN_375782393_400000_CN_155312475_400000/RConn2
  _CN_375782393_400000_CN_155312475_400000/RConn3 -- T_375782393__/LConn3 -- bus376/LConn1
  _CN_375782394_400000_CN_149865727_400000/RConn1 -- T_375782394__/LConn1 -- _CN_375782394_400000_CN_155312475_400000/RConn1
  _CN_375782394_400000_CN_149865727_400000/RConn2 -- T_375782394__/LConn2 -- _CN_375782394_400000_CN_155312475_400000/RConn2
  _CN_375782394_400000_CN_149865727_400000/RConn3 -- T_375782394__/LConn3 -- _CN_375782394_400000_CN_155312475_400000/RConn3 -- bus377/LConn1
  T_384824848__/RConn1 -- L_384824848/LConn1
  T_384824848__/RConn2 -- L_384824848/LConn2
  L_384824848/LConn3 -- T_384824848__/RConn3 -- bus378/LConn1
  T_115792106__/RConn1 -- L_115792106/LConn1
  T_115792106__/RConn2 -- L_115792106/LConn2
  L_115792106/LConn3 -- T_115792106__/RConn3 -- bus379/LConn1
  T_239626890__/RConn1 -- L_239626890/LConn1
  T_239626890__/RConn2 -- L_239626890/LConn2
  L_239626890/LConn3 -- T_239626890__/RConn3 -- bus380/LConn1
  T_384752553__/RConn1 -- L_384752553/LConn1
  T_384752553__/RConn2 -- L_384752553/LConn2
  L_384752553/LConn3 -- T_384752553__/RConn3 -- bus381/LConn1
  T_239679266__/RConn1 -- L_239679266/LConn1
  T_239679266__/RConn2 -- L_239679266/LConn2
  L_239679266/LConn3 -- T_239679266__/RConn3 -- bus382/LConn1
  T_384752846__/RConn1 -- L_384752846/LConn1
  T_384752846__/RConn2 -- L_384752846/LConn2
  L_384752846/LConn3 -- T_384752846__/RConn3 -- bus383/LConn1
  T_240050706__/RConn1 -- L_240050706/LConn1
  T_240050706__/RConn2 -- L_240050706/LConn2
  L_240050706/LConn3 -- T_240050706__/RConn3 -- bus384/LConn1
  T_240062607__/RConn1 -- L_240062607/LConn1
  T_240062607__/RConn2 -- L_240062607/LConn2
  L_240062607/LConn3 -- T_240062607__/RConn3 -- bus385/LConn1
  T_240045481__/RConn1 -- L_240045481/LConn1
  T_240045481__/RConn2 -- L_240045481/LConn2
  L_240045481/LConn3 -- T_240045481__/RConn3 -- bus386/LConn1
  T_242642583__/RConn1 -- L_242642583/LConn1
  T_242642583__/RConn2 -- L_242642583/LConn2
  L_242642583/LConn3 -- T_242642583__/RConn3 -- bus387/LConn1
  T_384800789__/RConn1 -- L_384800789/LConn1
  T_384800789__/RConn2 -- L_384800789/LConn2
  L_384800789/LConn3 -- T_384800789__/RConn3 -- bus388/LConn1
  T_115717271__/RConn1 -- L_115717271/LConn1
  T_115717271__/RConn2 -- L_115717271/LConn2
  L_115717271/LConn3 -- T_115717271__/RConn3 -- bus389/LConn1
  T_203617303__/RConn1 -- L_203617303/LConn1
  T_203617303__/RConn2 -- L_203617303/LConn2
  L_203617303/LConn3 -- T_203617303__/RConn3 -- bus390/LConn1
  T_203615053__/RConn1 -- L_203615053/LConn1
  T_203615053__/RConn2 -- L_203615053/LConn2
  L_203615053/LConn3 -- T_203615053__/RConn3 -- bus391/LConn1
  T_29499934__/RConn1 -- L_29499934/LConn1
  T_29499934__/RConn2 -- L_29499934/LConn2
  L_29499934/LConn3 -- T_29499934__/RConn3 -- bus392/LConn1
  T_354619026__/RConn1 -- L_354619026/LConn1
  T_354619026__/RConn2 -- L_354619026/LConn2
  L_354619026/LConn3 -- T_354619026__/RConn3 -- bus393/LConn1
  T_176665128__Substation_Kalba/RConn1 -- L_176665128/LConn1
  T_176665128__Substation_Kalba/RConn2 -- L_176665128/LConn2
  L_176665128/LConn3 -- T_176665128__Substation_Kalba/RConn3 -- bus394/LConn1
  T_220817213__substation_Al_Hayl/RConn1 -- L_220817213/LConn1
  T_220817213__substation_Al_Hayl/RConn2 -- L_220817213/LConn2
  L_220817213/LConn3 -- T_220817213__substation_Al_Hayl/RConn3 -- bus395/LConn1
  T_115205161__/RConn1 -- L_115205161/LConn1
  T_115205161__/RConn2 -- L_115205161/LConn2
  L_115205161/LConn3 -- T_115205161__/RConn3 -- bus396/LConn1
  T_52609391__/RConn1 -- L_52609391/LConn1
  T_52609391__/RConn2 -- L_52609391/LConn2
  L_52609391/LConn3 -- T_52609391__/RConn3 -- bus397/LConn1
  T_375782442__/RConn1 -- L_375782442/LConn1
  T_375782442__/RConn2 -- L_375782442/LConn2
  L_375782442/LConn3 -- T_375782442__/RConn3 -- bus398/LConn1
  T_386056423__/RConn1 -- L_386056423/LConn1
  T_386056423__/RConn2 -- L_386056423/LConn2
  L_386056423/LConn3 -- T_386056423__/RConn3 -- bus399/LConn1
  T_386056422__/RConn1 -- L_386056422/LConn1
  T_386056422__/RConn2 -- L_386056422/LConn2
  L_386056422/LConn3 -- T_386056422__/RConn3 -- bus400/LConn1
  T_232335918__/RConn1 -- L_232335918/LConn1
  T_232335918__/RConn2 -- L_232335918/LConn2
  L_232335918/LConn3 -- T_232335918__/RConn3 -- bus401/LConn1
  T_223140233__/RConn1 -- L_223140233/LConn1
  T_223140233__/RConn2 -- L_223140233/LConn2
  L_223140233/LConn3 -- T_223140233__/RConn3 -- bus402/LConn1
  T_39657769__/RConn1 -- L_39657769/LConn1
  T_39657769__/RConn2 -- L_39657769/LConn2
  L_39657769/LConn3 -- T_39657769__/RConn3 -- bus403/LConn1
  T_384714801__/RConn1 -- L_384714801/LConn1
  T_384714801__/RConn2 -- L_384714801/LConn2
  L_384714801/LConn3 -- T_384714801__/RConn3 -- bus404/LConn1
  T_386214966__/RConn1 -- L_386214966/LConn1
  T_386214966__/RConn2 -- L_386214966/LConn2
  L_386214966/LConn3 -- T_386214966__/RConn3 -- bus405/LConn1
  T_385548908__/RConn1 -- L_385548908/LConn1
  T_385548908__/RConn2 -- L_385548908/LConn2
  L_385548908/LConn3 -- T_385548908__/RConn3 -- bus406/LConn1
  T_60333463__/RConn1 -- L_60333463/LConn1
  T_60333463__/RConn2 -- L_60333463/LConn2
  L_60333463/LConn3 -- T_60333463__/RConn3 -- bus407/LConn1
  T_384714810__/RConn1 -- L_384714810/LConn1
  T_384714810__/RConn2 -- L_384714810/LConn2
  L_384714810/LConn3 -- T_384714810__/RConn3 -- bus408/LConn1
  T_385907829__/RConn1 -- L_385907829/LConn1
  T_385907829__/RConn2 -- L_385907829/LConn2
  L_385907829/LConn3 -- T_385907829__/RConn3 -- bus409/LConn1
  T_385907824__/RConn1 -- L_385907824/LConn1
  T_385907824__/RConn2 -- L_385907824/LConn2
  L_385907824/LConn3 -- T_385907824__/RConn3 -- bus410/LConn1
  T_173271221__/RConn1 -- L_173271221/LConn1
  T_173271221__/RConn2 -- L_173271221/LConn2
  L_173271221/LConn3 -- T_173271221__/RConn3 -- bus411/LConn1
  T_384714812__/RConn1 -- L_384714812/LConn1
  T_384714812__/RConn2 -- L_384714812/LConn2
  L_384714812/LConn3 -- T_384714812__/RConn3 -- bus412/LConn1
  T_240571747__/RConn1 -- L_240571747/LConn1
  T_240571747__/RConn2 -- L_240571747/LConn2
  L_240571747/LConn3 -- T_240571747__/RConn3 -- bus413/LConn1
  T_203985985__/RConn1 -- L_203985985/LConn1
  T_203985985__/RConn2 -- L_203985985/LConn2
  L_203985985/LConn3 -- T_203985985__/RConn3 -- bus414/LConn1
  T_203888070__/RConn1 -- L_203888070/LConn1
  T_203888070__/RConn2 -- L_203888070/LConn2
  L_203888070/LConn3 -- T_203888070__/RConn3 -- bus415/LConn1
  T_384961291__/RConn1 -- L_384961291/LConn1
  T_384961291__/RConn2 -- L_384961291/LConn2
  L_384961291/LConn3 -- T_384961291__/RConn3 -- bus416/LConn1
  T_94816858__/RConn1 -- L_94816858/LConn1
  T_94816858__/RConn2 -- L_94816858/LConn2
  L_94816858/LConn3 -- T_94816858__/RConn3 -- bus417/LConn1
  T_384961303__/RConn1 -- L_384961303/LConn1
  T_384961303__/RConn2 -- L_384961303/LConn2
  L_384961303/LConn3 -- T_384961303__/RConn3 -- bus418/LConn1
  T_384961300__/RConn1 -- L_384961300/LConn1
  T_384961300__/RConn2 -- L_384961300/LConn2
  L_384961300/LConn3 -- T_384961300__/RConn3 -- bus419/LConn1
  T_328560711__/RConn1 -- L_328560711/LConn1
  T_328560711__/RConn2 -- L_328560711/LConn2
  L_328560711/LConn3 -- T_328560711__/RConn3 -- bus420/LConn1
  T_123775127__/RConn1 -- L_123775127/LConn1
  T_123775127__/RConn2 -- L_123775127/LConn2
  L_123775127/LConn3 -- T_123775127__/RConn3 -- bus421/LConn1
  T_168770199__/RConn1 -- L_168770199/LConn1
  T_168770199__/RConn2 -- L_168770199/LConn2
  L_168770199/LConn3 -- T_168770199__/RConn3 -- bus422/LConn1
  T_132132424__/RConn1 -- L_132132424/LConn1
  T_132132424__/RConn2 -- L_132132424/LConn2
  L_132132424/LConn3 -- T_132132424__/RConn3 -- bus423/LConn1
  T_132154026__/RConn1 -- L_132154026/LConn1
  T_132154026__/RConn2 -- L_132154026/LConn2
  L_132154026/LConn3 -- T_132154026__/RConn3 -- bus424/LConn1
  T_112321201__substation/RConn1 -- L_112321201/LConn1
  T_112321201__substation/RConn2 -- L_112321201/LConn2
  L_112321201/LConn3 -- T_112321201__substation/RConn3 -- bus425/LConn1
  T_112521127__substation/RConn1 -- L_112521127/LConn1
  T_112521127__substation/RConn2 -- L_112521127/LConn2
  L_112521127/LConn3 -- T_112521127__substation/RConn3 -- bus426/LConn1
  T_122262836__/RConn1 -- L_122262836/LConn1
  T_122262836__/RConn2 -- L_122262836/LConn2
  L_122262836/LConn3 -- T_122262836__/RConn3 -- bus427/LConn1
  T_239976013__/RConn1 -- L_239976013/LConn1
  T_239976013__/RConn2 -- L_239976013/LConn2
  L_239976013/LConn3 -- T_239976013__/RConn3 -- bus428/LConn1
  T_239939959__/RConn1 -- L_239939959/LConn1
  T_239939959__/RConn2 -- L_239939959/LConn2
  L_239939959/LConn3 -- T_239939959__/RConn3 -- bus429/LConn1
  T_239937124__/RConn1 -- L_239937124/LConn1
  T_239937124__/RConn2 -- L_239937124/LConn2
  L_239937124/LConn3 -- T_239937124__/RConn3 -- bus430/LConn1
  T_384684174__/RConn1 -- L_384684174/LConn1
  T_384684174__/RConn2 -- L_384684174/LConn2
  L_384684174/LConn3 -- T_384684174__/RConn3 -- bus431/LConn1
  T_115717711__/RConn1 -- L_115717711/LConn1
  T_115717711__/RConn2 -- L_115717711/LConn2
  L_115717711/LConn3 -- T_115717711__/RConn3 -- bus432/LConn1
  T_115797297__/RConn1 -- L_115797297/LConn1
  T_115797297__/RConn2 -- L_115797297/LConn2
  L_115797297/LConn3 -- T_115797297__/RConn3 -- bus433/LConn1
  T_115797291__/RConn1 -- L_115797291/LConn1
  T_115797291__/RConn2 -- L_115797291/LConn2
  L_115797291/LConn3 -- T_115797291__/RConn3 -- bus434/LConn1
  T_242205776__/RConn1 -- L_242205776/LConn1
  T_242205776__/RConn2 -- L_242205776/LConn2
  L_242205776/LConn3 -- T_242205776__/RConn3 -- bus435/LConn1
  T_242166513__/RConn1 -- L_242166513/LConn1
  T_242166513__/RConn2 -- L_242166513/LConn2
  L_242166513/LConn3 -- T_242166513__/RConn3 -- bus436/LConn1
  T_239581995__/RConn1 -- L_239581995/LConn1
  T_239581995__/RConn2 -- L_239581995/LConn2
  L_239581995/LConn3 -- T_239581995__/RConn3 -- bus437/LConn1
  T_384753595__/RConn1 -- L_384753595/LConn1
  T_384753595__/RConn2 -- L_384753595/LConn2
  L_384753595/LConn3 -- T_384753595__/RConn3 -- bus438/LConn1
  T_384911487__/RConn1 -- L_384911487/LConn1
  T_384911487__/RConn2 -- L_384911487/LConn2
  L_384911487/LConn3 -- T_384911487__/RConn3 -- bus439/LConn1
  T_353897470__/RConn1 -- L_353897470/LConn1
  T_353897470__/RConn2 -- L_353897470/LConn2
  L_353897470/LConn3 -- T_353897470__/RConn3 -- bus440/LConn1
  T_242205780__/RConn1 -- L_242205780/LConn1
  T_242205780__/RConn2 -- L_242205780/LConn2
  L_242205780/LConn3 -- T_242205780__/RConn3 -- bus441/LConn1
  T_94816849__/RConn1 -- L_94816849/LConn1
  T_94816849__/RConn2 -- L_94816849/LConn2
  L_94816849/LConn3 -- T_94816849__/RConn3 -- bus442/LConn1
  T_181332831__/RConn1 -- L_181332831/LConn1
  T_181332831__/RConn2 -- L_181332831/LConn2
  L_181332831/LConn3 -- T_181332831__/RConn3 -- bus443/LConn1
  T_240571748__/RConn1 -- L_240571748/LConn1
  T_240571748__/RConn2 -- L_240571748/LConn2
  L_240571748/LConn3 -- T_240571748__/RConn3 -- bus444/LConn1
  T_204266069__/RConn1 -- L_204266069/LConn1
  T_204266069__/RConn2 -- L_204266069/LConn2
  L_204266069/LConn3 -- T_204266069__/RConn3 -- bus445/LConn1
  T_204267684__/RConn1 -- L_204267684/LConn1
  T_204267684__/RConn2 -- L_204267684/LConn2
  L_204267684/LConn3 -- T_204267684__/RConn3 -- bus446/LConn1
  T_204553547__substation/RConn1 -- L_204553547/LConn1
  T_204553547__substation/RConn2 -- L_204553547/LConn2
  L_204553547/LConn3 -- T_204553547__substation/RConn3 -- bus447/LConn1
  T_146511548__/RConn1 -- L_146511548/LConn1
  T_146511548__/RConn2 -- L_146511548/LConn2
  L_146511548/LConn3 -- T_146511548__/RConn3 -- bus448/LConn1
  T_242539627__/RConn1 -- L_242539627/LConn1
  T_242539627__/RConn2 -- L_242539627/LConn2
  L_242539627/LConn3 -- T_242539627__/RConn3 -- bus449/LConn1
  T_239435500__/RConn1 -- L_239435500/LConn1
  T_239435500__/RConn2 -- L_239435500/LConn2
  L_239435500/LConn3 -- T_239435500__/RConn3 -- bus450/LConn1
  T_386200252__/RConn1 -- L_386200252/LConn1
  T_386200252__/RConn2 -- L_386200252/LConn2
  L_386200252/LConn3 -- T_386200252__/RConn3 -- bus451/LConn1
  T_60333184__/RConn1 -- L_60333184/LConn1
  T_60333184__/RConn2 -- L_60333184/LConn2
  L_60333184/LConn3 -- T_60333184__/RConn3 -- bus452/LConn1
  T_384708869__/RConn1 -- L_384708869/LConn1
  T_384708869__/RConn2 -- L_384708869/LConn2
  L_384708869/LConn3 -- T_384708869__/RConn3 -- bus453/LConn1
  T_239946325__/RConn1 -- L_239946325/LConn1
  T_239946325__/RConn2 -- L_239946325/LConn2
  L_239946325/LConn3 -- T_239946325__/RConn3 -- bus454/LConn1
  T_354672637__/RConn1 -- L_354672637/LConn1
  T_354672637__/RConn2 -- L_354672637/LConn2
  L_354672637/LConn3 -- T_354672637__/RConn3 -- bus455/LConn1
  T_386200253__/RConn1 -- L_386200253/LConn1
  T_386200253__/RConn2 -- L_386200253/LConn2
  L_386200253/LConn3 -- T_386200253__/RConn3 -- bus456/LConn1
  T_39657770__/RConn1 -- L_39657770/LConn1
  T_39657770__/RConn2 -- L_39657770/LConn2
  L_39657770/LConn3 -- T_39657770__/RConn3 -- bus457/LConn1
  T_385907825__/RConn1 -- L_385907825/LConn1
  T_385907825__/RConn2 -- L_385907825/LConn2
  L_385907825/LConn3 -- T_385907825__/RConn3 -- bus458/LConn1
  T_385907834__/RConn1 -- L_385907834/LConn1
  T_385907834__/RConn2 -- L_385907834/LConn2
  L_385907834/LConn3 -- T_385907834__/RConn3 -- bus459/LConn1
  T_384902258__/RConn1 -- L_384902258/LConn1
  T_384902258__/RConn2 -- L_384902258/LConn2
  L_384902258/LConn3 -- T_384902258__/RConn3 -- bus460/LConn1
  T_354672633__/RConn1 -- L_354672633/LConn1
  T_354672633__/RConn2 -- L_354672633/LConn2
  L_354672633/LConn3 -- T_354672633__/RConn3 -- bus461/LConn1
  T_240196788__/RConn1 -- L_240196788/LConn1
  T_240196788__/RConn2 -- L_240196788/LConn2
  L_240196788/LConn3 -- T_240196788__/RConn3 -- bus462/LConn1
  T_384902262__/RConn1 -- L_384902262/LConn1
  T_384902262__/RConn2 -- L_384902262/LConn2
  L_384902262/LConn3 -- T_384902262__/RConn3 -- bus463/LConn1
  T_112460404__/RConn1 -- L_112460404/LConn1
  T_112460404__/RConn2 -- L_112460404/LConn2
  L_112460404/LConn3 -- T_112460404__/RConn3 -- bus464/LConn1
  T_295186316__/RConn1 -- L_295186316/LConn1
  T_295186316__/RConn2 -- L_295186316/LConn2
  L_295186316/LConn3 -- T_295186316__/RConn3 -- bus465/LConn1
  T_112460405__/RConn1 -- L_112460405/LConn1
  T_112460405__/RConn2 -- L_112460405/LConn2
  L_112460405/LConn3 -- T_112460405__/RConn3 -- bus466/LConn1
  T_199776373__/RConn1 -- L_199776373/LConn1
  T_199776373__/RConn2 -- L_199776373/LConn2
  L_199776373/LConn3 -- T_199776373__/RConn3 -- bus467/LConn1
  T_239687287__/RConn1 -- L_239687287/LConn1
  T_239687287__/RConn2 -- L_239687287/LConn2
  L_239687287/LConn3 -- T_239687287__/RConn3 -- bus468/LConn1
  T_239694763__/RConn1 -- L_239694763/LConn1
  T_239694763__/RConn2 -- L_239694763/LConn2
  L_239694763/LConn3 -- T_239694763__/RConn3 -- bus469/LConn1
  T_223684728__/RConn1 -- L_223684728/LConn1
  T_223684728__/RConn2 -- L_223684728/LConn2
  L_223684728/LConn3 -- T_223684728__/RConn3 -- bus470/LConn1
  T_379753822__/RConn1 -- L_379753822/LConn1
  T_379753822__/RConn2 -- L_379753822/LConn2
  L_379753822/LConn3 -- T_379753822__/RConn3 -- bus471/LConn1
  T_424681663__/RConn1 -- L_424681663/LConn1
  T_424681663__/RConn2 -- L_424681663/LConn2
  L_424681663/LConn3 -- T_424681663__/RConn3 -- bus472/LConn1
  T_424681664__/RConn1 -- L_424681664/LConn1
  T_424681664__/RConn2 -- L_424681664/LConn2
  L_424681664/LConn3 -- T_424681664__/RConn3 -- bus473/LConn1
  T_168549720__/RConn1 -- L_168549720/LConn1
  T_168549720__/RConn2 -- L_168549720/LConn2
  L_168549720/LConn3 -- T_168549720__/RConn3 -- bus474/LConn1
  T_385113219__/RConn1 -- L_385113219/LConn1
  T_385113219__/RConn2 -- L_385113219/LConn2
  L_385113219/LConn3 -- T_385113219__/RConn3 -- bus475/LConn1
  T_227922803__/RConn1 -- L_227922803/LConn1
  T_227922803__/RConn2 -- L_227922803/LConn2
  L_227922803/LConn3 -- T_227922803__/RConn3 -- bus476/LConn1
  T_94816976__/RConn1 -- L_94816976/LConn1
  T_94816976__/RConn2 -- L_94816976/LConn2
  L_94816976/LConn3 -- T_94816976__/RConn3 -- bus477/LConn1
  T_384684166__/RConn1 -- L_384684166/LConn1
  T_384684166__/RConn2 -- L_384684166/LConn2
  L_384684166/LConn3 -- T_384684166__/RConn3 -- bus478/LConn1
  T_239990687__/RConn1 -- L_239990687/LConn1
  T_239990687__/RConn2 -- L_239990687/LConn2
  L_239990687/LConn3 -- T_239990687__/RConn3 -- bus479/LConn1
  T_240000160__/RConn1 -- L_240000160/LConn1
  T_240000160__/RConn2 -- L_240000160/LConn2
  L_240000160/LConn3 -- T_240000160__/RConn3 -- bus480/LConn1
  T_239990697__/RConn1 -- L_239990697/LConn1
  T_239990697__/RConn2 -- L_239990697/LConn2
  L_239990697/LConn3 -- T_239990697__/RConn3 -- bus481/LConn1
  T_115677406__/RConn1 -- L_115677406/LConn1
  T_115677406__/RConn2 -- L_115677406/LConn2
  L_115677406/LConn3 -- T_115677406__/RConn3 -- bus482/LConn1
  T_384908661__/RConn1 -- L_384908661/LConn1
  T_384908661__/RConn2 -- L_384908661/LConn2
  L_384908661/LConn3 -- T_384908661__/RConn3 -- bus483/LConn1
  T_115717268__/RConn1 -- L_115717268/LConn1
  T_115717268__/RConn2 -- L_115717268/LConn2
  L_115717268/LConn3 -- T_115717268__/RConn3 -- bus484/LConn1
  T_115717276__/RConn1 -- L_115717276/LConn1
  T_115717276__/RConn2 -- L_115717276/LConn2
  L_115717276/LConn3 -- T_115717276__/RConn3 -- bus485/LConn1
  T_115717269__/RConn1 -- L_115717269/LConn1
  T_115717269__/RConn2 -- L_115717269/LConn2
  L_115717269/LConn3 -- T_115717269__/RConn3 -- bus486/LConn1
  T_115717275__/RConn1 -- L_115717275/LConn1
  T_115717275__/RConn2 -- L_115717275/LConn2
  L_115717275/LConn3 -- T_115717275__/RConn3 -- bus487/LConn1
  T_189281434__/RConn1 -- L_189281434/LConn1
  T_189281434__/RConn2 -- L_189281434/LConn2
  L_189281434/LConn3 -- T_189281434__/RConn3 -- bus488/LConn1
  T_168190854__/RConn1 -- L_168190854/LConn1
  T_168190854__/RConn2 -- L_168190854/LConn2
  L_168190854/LConn3 -- T_168190854__/RConn3 -- bus489/LConn1
  T_94816929__/RConn1 -- L_94816929/LConn1
  T_94816929__/RConn2 -- L_94816929/LConn2
  L_94816929/LConn3 -- T_94816929__/RConn3 -- bus490/LConn1
  T_173919914__/RConn1 -- L_173919914/LConn1
  T_173919914__/RConn2 -- L_173919914/LConn2
  L_173919914/LConn3 -- T_173919914__/RConn3 -- bus491/LConn1
  T_204142303__/RConn1 -- L_204142303/LConn1
  T_204142303__/RConn2 -- L_204142303/LConn2
  L_204142303/LConn3 -- T_204142303__/RConn3 -- bus492/LConn1
  T_385263258__/RConn1 -- L_385263258/LConn1
  T_385263258__/RConn2 -- L_385263258/LConn2
  L_385263258/LConn3 -- T_385263258__/RConn3 -- bus493/LConn1
  T_298351271__/RConn1 -- L_298351271/LConn1
  T_298351271__/RConn2 -- L_298351271/LConn2
  L_298351271/LConn3 -- T_298351271__/RConn3 -- bus494/LConn1
  T_133861049__/RConn1 -- L_133861049/LConn1
  T_133861049__/RConn2 -- L_133861049/LConn2
  L_133861049/LConn3 -- T_133861049__/RConn3 -- bus495/LConn1
  T_133861050__/RConn1 -- L_133861050/LConn1
  T_133861050__/RConn2 -- L_133861050/LConn2
  L_133861050/LConn3 -- T_133861050__/RConn3 -- bus496/LConn1
  T_384822726__/RConn1 -- L_384822726/LConn1
  T_384822726__/RConn2 -- L_384822726/LConn2
  L_384822726/LConn3 -- T_384822726__/RConn3 -- bus497/LConn1
  T_385113202__/RConn1 -- L_385113202/LConn1
  T_385113202__/RConn2 -- L_385113202/LConn2
  L_385113202/LConn3 -- T_385113202__/RConn3 -- bus498/LConn1
  T_94816975__/RConn1 -- L_94816975/LConn1
  T_94816975__/RConn2 -- L_94816975/LConn2
  L_94816975/LConn3 -- T_94816975__/RConn3 -- bus499/LConn1
  T_133865685__/RConn1 -- L_133865685/LConn1
  T_133865685__/RConn2 -- L_133865685/LConn2
  L_133865685/LConn3 -- T_133865685__/RConn3 -- bus500/LConn1
  T_242544315__/RConn1 -- L_242544315/LConn1
  T_242544315__/RConn2 -- L_242544315/LConn2
  L_242544315/LConn3 -- T_242544315__/RConn3 -- bus501/LConn1
  T_384708877__/RConn1 -- L_384708877/LConn1
  T_384708877__/RConn2 -- L_384708877/LConn2
  L_384708877/LConn3 -- T_384708877__/RConn3 -- bus502/LConn1
  T_384708875__/RConn1 -- L_384708875/LConn1
  T_384708875__/RConn2 -- L_384708875/LConn2
  L_384708875/LConn3 -- T_384708875__/RConn3 -- bus503/LConn1
  T_243443456__/RConn1 -- L_243443456/LConn1
  T_243443456__/RConn2 -- L_243443456/LConn2
  L_243443456/LConn3 -- T_243443456__/RConn3 -- bus504/LConn1
  T_385086141__/RConn1 -- L_385086141/LConn1
  T_385086141__/RConn2 -- L_385086141/LConn2
  L_385086141/LConn3 -- T_385086141__/RConn3 -- bus505/LConn1
  T_424681656__/RConn1 -- L_424681656/LConn1
  T_424681656__/RConn2 -- L_424681656/LConn2
  L_424681656/LConn3 -- T_424681656__/RConn3 -- bus506/LConn1
  T_201082863__/RConn1 -- L_201082863/LConn1
  T_201082863__/RConn2 -- L_201082863/LConn2
  L_201082863/LConn3 -- T_201082863__/RConn3 -- bus507/LConn1
  T_115677382__/RConn1 -- L_115677382/LConn1
  T_115677382__/RConn2 -- L_115677382/LConn2
  L_115677382/LConn3 -- T_115677382__/RConn3 -- bus508/LConn1
  T_115677394__/RConn1 -- L_115677394/LConn1
  T_115677394__/RConn2 -- L_115677394/LConn2
  L_115677394/LConn3 -- T_115677394__/RConn3 -- bus509/LConn1
  T_115677404__/RConn1 -- L_115677404/LConn1
  T_115677404__/RConn2 -- L_115677404/LConn2
  L_115677404/LConn3 -- T_115677404__/RConn3 -- bus510/LConn1
  T_354672638__/RConn1 -- L_354672638/LConn1
  T_354672638__/RConn2 -- L_354672638/LConn2
  L_354672638/LConn3 -- T_354672638__/RConn3 -- bus511/LConn1
  T_354672635__/RConn1 -- L_354672635/LConn1
  T_354672635__/RConn2 -- L_354672635/LConn2
  L_354672635/LConn3 -- T_354672635__/RConn3 -- bus512/LConn1
  T_203614925__/RConn1 -- L_203614925/LConn1
  T_203614925__/RConn2 -- L_203614925/LConn2
  L_203614925/LConn3 -- T_203614925__/RConn3 -- bus513/LConn1
  T_303315256__/RConn1 -- L_303315256/LConn1
  T_303315256__/RConn2 -- L_303315256/LConn2
  L_303315256/LConn3 -- T_303315256__/RConn3 -- bus514/LConn1
  T_303315257__/RConn1 -- L_303315257/LConn1
  T_303315257__/RConn2 -- L_303315257/LConn2
  L_303315257/LConn3 -- T_303315257__/RConn3 -- bus515/LConn1
  T_115305410__/RConn1 -- L_115305410/LConn1
  T_115305410__/RConn2 -- L_115305410/LConn2
  L_115305410/LConn3 -- T_115305410__/RConn3 -- bus516/LConn1
  T_203979987__/RConn1 -- L_203979987/LConn1
  T_203979987__/RConn2 -- L_203979987/LConn2
  L_203979987/LConn3 -- T_203979987__/RConn3 -- bus517/LConn1
  T_115188435__/RConn1 -- L_115188435/LConn1
  T_115188435__/RConn2 -- L_115188435/LConn2
  L_115188435/LConn3 -- T_115188435__/RConn3 -- bus518/LConn1
  T_115204753__/RConn1 -- L_115204753/LConn1
  T_115204753__/RConn2 -- L_115204753/LConn2
  L_115204753/LConn3 -- T_115204753__/RConn3 -- bus519/LConn1
  T_219620566__substation/RConn1 -- L_219620566/LConn1
  T_219620566__substation/RConn2 -- L_219620566/LConn2
  L_219620566/LConn3 -- T_219620566__substation/RConn3 -- bus520/LConn1
  T_295186319__/RConn1 -- L_295186319/LConn1
  T_295186319__/RConn2 -- L_295186319/LConn2
  L_295186319/LConn3 -- T_295186319__/RConn3 -- bus521/LConn1
  T_181332857__/RConn1 -- L_181332857/LConn1
  T_181332857__/RConn2 -- L_181332857/LConn2
  L_181332857/LConn3 -- T_181332857__/RConn3 -- bus522/LConn1
  T_181332751__/RConn1 -- L_181332751/LConn1
  T_181332751__/RConn2 -- L_181332751/LConn2
  L_181332751/LConn3 -- T_181332751__/RConn3 -- bus523/LConn1
  T_204141035__/RConn1 -- L_204141035/LConn1
  T_204141035__/RConn2 -- L_204141035/LConn2
  L_204141035/LConn3 -- T_204141035__/RConn3 -- bus524/LConn1
  T_115677419__/RConn1 -- L_115677419/LConn1
  T_115677419__/RConn2 -- L_115677419/LConn2
  L_115677419/LConn3 -- T_115677419__/RConn3 -- bus525/LConn1
  T_386138424__/RConn1 -- L_386138424/LConn1
  T_386138424__/RConn2 -- L_386138424/LConn2
  L_386138424/LConn3 -- T_386138424__/RConn3 -- bus526/LConn1
  T_385629058__/RConn1 -- L_385629058/LConn1
  T_385629058__/RConn2 -- L_385629058/LConn2
  L_385629058/LConn3 -- T_385629058__/RConn3 -- bus527/LConn1
  T_386202923__/RConn1 -- L_386202923/LConn1
  T_386202923__/RConn2 -- L_386202923/LConn2
  L_386202923/LConn3 -- T_386202923__/RConn3 -- bus528/LConn1
  T_216208125__/RConn1 -- L_216208125/LConn1
  T_216208125__/RConn2 -- L_216208125/LConn2
  L_216208125/LConn3 -- T_216208125__/RConn3 -- bus529/LConn1
  T_115310393__/RConn1 -- L_115310393/LConn1
  T_115310393__/RConn2 -- L_115310393/LConn2
  L_115310393/LConn3 -- T_115310393__/RConn3 -- bus530/LConn1
  T_240323330__/RConn1 -- L_240323330/LConn1
  T_240323330__/RConn2 -- L_240323330/LConn2
  L_240323330/LConn3 -- T_240323330__/RConn3 -- bus531/LConn1
  T_215091971__/RConn1 -- L_215091971/LConn1
  T_215091971__/RConn2 -- L_215091971/LConn2
  L_215091971/LConn3 -- T_215091971__/RConn3 -- bus532/LConn1
  T_215091972__/RConn1 -- L_215091972/LConn1
  T_215091972__/RConn2 -- L_215091972/LConn2
  L_215091972/LConn3 -- T_215091972__/RConn3 -- bus533/LConn1
  T_386063272__/RConn1 -- L_386063272/LConn1
  T_386063272__/RConn2 -- L_386063272/LConn2
  L_386063272/LConn3 -- T_386063272__/RConn3 -- bus534/LConn1
  T_240292205__/RConn1 -- L_240292205/LConn1
  T_240292205__/RConn2 -- L_240292205/LConn2
  L_240292205/LConn3 -- T_240292205__/RConn3 -- bus535/LConn1
  T_240292204__/RConn1 -- L_240292204/LConn1
  T_240292204__/RConn2 -- L_240292204/LConn2
  L_240292204/LConn3 -- T_240292204__/RConn3 -- bus536/LConn1
  T_239679334__/RConn1 -- L_239679334/LConn1
  T_239679334__/RConn2 -- L_239679334/LConn2
  L_239679334/LConn3 -- T_239679334__/RConn3 -- bus537/LConn1
  T_39657768__/RConn1 -- L_39657768/LConn1
  T_39657768__/RConn2 -- L_39657768/LConn2
  L_39657768/LConn3 -- T_39657768__/RConn3 -- bus538/LConn1
  T_115797300__/RConn1 -- L_115797300/LConn1
  T_115797300__/RConn2 -- L_115797300/LConn2
  L_115797300/LConn3 -- T_115797300__/RConn3 -- bus539/LConn1
  T_385499970__/RConn1 -- L_385499970/LConn1
  T_385499970__/RConn2 -- L_385499970/LConn2
  L_385499970/LConn3 -- T_385499970__/RConn3 -- bus540/LConn1
  T_203975634__/RConn1 -- L_203975634/LConn1
  T_203975634__/RConn2 -- L_203975634/LConn2
  L_203975634/LConn3 -- T_203975634__/RConn3 -- bus541/LConn1
  T_369326404__/RConn1 -- L_369326404/LConn1
  T_369326404__/RConn2 -- L_369326404/LConn2
  L_369326404/LConn3 -- T_369326404__/RConn3 -- bus542/LConn1
  T_190221972__/RConn1 -- L_190221972/LConn1
  T_190221972__/RConn2 -- L_190221972/LConn2
  L_190221972/LConn3 -- T_190221972__/RConn3 -- bus543/LConn1
  T_240577351__/RConn1 -- L_240577351/LConn1
  T_240577351__/RConn2 -- L_240577351/LConn2
  L_240577351/LConn3 -- T_240577351__/RConn3 -- bus544/LConn1
  T_384716522__/RConn1 -- L_384716522/LConn1
  T_384716522__/RConn2 -- L_384716522/LConn2
  L_384716522/LConn3 -- T_384716522__/RConn3 -- bus545/LConn1
  T_168661559__/RConn1 -- L_168661559/LConn1
  T_168661559__/RConn2 -- L_168661559/LConn2
  L_168661559/LConn3 -- T_168661559__/RConn3 -- bus546/LConn1
  T_188636744__/RConn1 -- L_188636744/LConn1
  T_188636744__/RConn2 -- L_188636744/LConn2
  L_188636744/LConn3 -- T_188636744__/RConn3 -- bus547/LConn1
  T_386208076__/RConn1 -- L_386208076/LConn1
  T_386208076__/RConn2 -- L_386208076/LConn2
  L_386208076/LConn3 -- T_386208076__/RConn3 -- bus548/LConn1
  T_181133259__/RConn1 -- L_181133259/LConn1
  T_181133259__/RConn2 -- L_181133259/LConn2
  L_181133259/LConn3 -- T_181133259__/RConn3 -- bus549/LConn1
  T_167842250__/RConn1 -- L_167842250/LConn1
  T_167842250__/RConn2 -- L_167842250/LConn2
  L_167842250/LConn3 -- T_167842250__/RConn3 -- bus550/LConn1
  T_384688538__/RConn1 -- L_384688538/LConn1
  T_384688538__/RConn2 -- L_384688538/LConn2
  L_384688538/LConn3 -- T_384688538__/RConn3 -- bus551/LConn1
  T_181132699__/RConn1 -- L_181132699/LConn1
  T_181132699__/RConn2 -- L_181132699/LConn2
  L_181132699/LConn3 -- T_181132699__/RConn3 -- bus552/LConn1
  T_384688544__/RConn1 -- L_384688544/LConn1
  T_384688544__/RConn2 -- L_384688544/LConn2
  L_384688544/LConn3 -- T_384688544__/RConn3 -- bus553/LConn1
  T_384731081__/RConn1 -- L_384731081/LConn1
  T_384731081__/RConn2 -- L_384731081/LConn2
  L_384731081/LConn3 -- T_384731081__/RConn3 -- bus554/LConn1
  T_199713782__/RConn1 -- L_199713782/LConn1
  T_199713782__/RConn2 -- L_199713782/LConn2
  L_199713782/LConn3 -- T_199713782__/RConn3 -- bus555/LConn1
  T_29504133__Substation/RConn1 -- L_29504133/LConn1
  T_29504133__Substation/RConn2 -- L_29504133/LConn2
  L_29504133/LConn3 -- T_29504133__Substation/RConn3 -- bus556/LConn1
  T_94950857__/RConn1 -- L_94950857/LConn1
  T_94950857__/RConn2 -- L_94950857/LConn2
  L_94950857/LConn3 -- T_94950857__/RConn3 -- bus557/LConn1
  T_95046332__Mussafah_GIC_Substation/RConn1 -- L_95046332/LConn1
  T_95046332__Mussafah_GIC_Substation/RConn2 -- L_95046332/LConn2
  L_95046332/LConn3 -- T_95046332__Mussafah_GIC_Substation/RConn3 -- bus558/LConn1
  T_29503687__Substation/RConn1 -- L_29503687/LConn1
  T_29503687__Substation/RConn2 -- L_29503687/LConn2
  L_29503687/LConn3 -- T_29503687__Substation/RConn3 -- bus559/LConn1
  T_95046964__Khazna/RConn1 -- L_95046964/LConn1
  T_95046964__Khazna/RConn2 -- L_95046964/LConn2
  L_95046964/LConn3 -- T_95046964__Khazna/RConn3 -- bus560/LConn1
  T_95084794__/RConn1 -- L_95084794/LConn1
  T_95084794__/RConn2 -- L_95084794/LConn2
  L_95084794/LConn3 -- T_95084794__/RConn3 -- bus561/LConn1
  T_95055625__Ramah/RConn1 -- L_95055625/LConn1
  T_95055625__Ramah/RConn2 -- L_95055625/LConn2
  L_95055625/LConn3 -- T_95055625__Ramah/RConn3 -- bus562/LConn1
  T_95084816__/RConn1 -- L_95084816/LConn1
  T_95084816__/RConn2 -- L_95084816/LConn2
  L_95084816/LConn3 -- T_95084816__/RConn3 -- bus563/LConn1
  T_200057688__AASW/RConn1 -- L_200057688/LConn1
  T_200057688__AASW/RConn2 -- L_200057688/LConn2
  L_200057688/LConn3 -- T_200057688__AASW/RConn3 -- bus564/LConn1
  T_95097245__Al_Wagon/RConn1 -- L_95097245/LConn1
  T_95097245__Al_Wagon/RConn2 -- L_95097245/LConn2
  L_95097245/LConn3 -- T_95097245__Al_Wagon/RConn3 -- bus565/LConn1
  T_95084811__Arad/RConn1 -- L_95084811/LConn1
  T_95084811__Arad/RConn2 -- L_95084811/LConn2
  L_95084811/LConn3 -- T_95084811__Arad/RConn3 -- bus566/LConn1
  T_132159924__Umm_Al_Oush/RConn1 -- L_132159924/LConn1
  T_132159924__Umm_Al_Oush/RConn2 -- L_132159924/LConn2
  L_132159924/LConn3 -- T_132159924__Umm_Al_Oush/RConn3 -- bus567/LConn1
  T_29500305__/RConn1 -- L_29500305/LConn1
  T_29500305__/RConn2 -- L_29500305/LConn2
  L_29500305/LConn3 -- T_29500305__/RConn3 -- bus568/LConn1
  T_181362976__Substation/RConn1 -- L_181362976/LConn1
  T_181362976__Substation/RConn2 -- L_181362976/LConn2
  L_181362976/LConn3 -- T_181362976__Substation/RConn3 -- bus569/LConn1
  T_95084771__/RConn1 -- L_95084771/LConn1
  T_95084771__/RConn2 -- L_95084771/LConn2
  L_95084771/LConn3 -- T_95084771__/RConn3 -- bus570/LConn1
  T_95097252__Dabiya/RConn1 -- L_95097252/LConn1
  T_95097252__Dabiya/RConn2 -- L_95097252/LConn2
  L_95097252/LConn3 -- T_95097252__Dabiya/RConn3 -- bus571/LConn1
  T_181332765__Central/RConn1 -- L_181332765/LConn1
  T_181332765__Central/RConn2 -- L_181332765/LConn2
  L_181332765/LConn3 -- T_181332765__Central/RConn3 -- bus572/LConn1
  T_95084776__/RConn1 -- L_95084776/LConn1
  T_95084776__/RConn2 -- L_95084776/LConn2
  L_95084776/LConn3 -- T_95084776__/RConn3 -- bus573/LConn1
  T_354672631__/RConn1 -- L_354672631/LConn1
  T_354672631__/RConn2 -- L_354672631/LConn2
  L_354672631/LConn3 -- T_354672631__/RConn3 -- bus574/LConn1
  T_215795245__Rumaithy/RConn1 -- L_215795245/LConn1
  T_215795245__Rumaithy/RConn2 -- L_215795245/LConn2
  L_215795245/LConn3 -- T_215795245__Rumaithy/RConn3 -- bus575/LConn1
  T_181361589__Asab/RConn1 -- L_181361589/LConn1
  T_181361589__Asab/RConn2 -- L_181361589/LConn2
  L_181361589/LConn3 -- T_181361589__Asab/RConn3 -- bus576/LConn1
  T_95099964__Madinat_Zayed/RConn1 -- L_95099964/LConn1
  T_95099964__Madinat_Zayed/RConn2 -- L_95099964/LConn2
  L_95099964/LConn3 -- T_95099964__Madinat_Zayed/RConn3 -- bus577/LConn1
  T_132159930__Sila/RConn1 -- L_132159930/LConn1
  T_132159930__Sila/RConn2 -- L_132159930/LConn2
  L_132159930/LConn3 -- T_132159930__Sila/RConn3 -- bus578/LConn1
  T_132517028__Ruwais/RConn1 -- L_132517028/LConn1
  T_132517028__Ruwais/RConn2 -- L_132517028/LConn2
  L_132517028/LConn3 -- T_132517028__Ruwais/RConn3 -- bus579/LConn1
  T_247122500__/RConn1 -- L_247122500/LConn1
  T_247122500__/RConn2 -- L_247122500/LConn2
  L_247122500/LConn3 -- T_247122500__/RConn3 -- bus580/LConn1
  T_95099973__Liwa/RConn1 -- L_95099973/LConn1
  T_95099973__Liwa/RConn2 -- L_95099973/LConn2
  L_95099973/LConn3 -- T_95099973__Liwa/RConn3 -- bus581/LConn1
  T_115677398__/RConn1 -- L_115677398/LConn1
  T_115677398__/RConn2 -- L_115677398/LConn2
  L_115677398/LConn3 -- T_115677398__/RConn3 -- bus582/LConn1
  T_386199534__/RConn1 -- L_386199534/LConn1
  T_386199534__/RConn2 -- L_386199534/LConn2
  L_386199534/LConn3 -- T_386199534__/RConn3 -- bus583/LConn1
  T_95084793__/RConn1 -- L_95084793/LConn1
  T_95084793__/RConn2 -- L_95084793/LConn2
  L_95084793/LConn3 -- T_95084793__/RConn3 -- bus584/LConn1
  T_386199541__/RConn1 -- L_386199541/LConn1
  T_386199541__/RConn2 -- L_386199541/LConn2
  L_386199541/LConn3 -- T_386199541__/RConn3 -- bus585/LConn1
  T_198365955__/RConn1 -- L_198365955/LConn1
  T_198365955__/RConn2 -- L_198365955/LConn2
  L_198365955/LConn3 -- T_198365955__/RConn3 -- bus586/LConn1
  T_199091189__/RConn1 -- L_199091189/LConn1
  T_199091189__/RConn2 -- L_199091189/LConn2
  L_199091189/LConn3 -- T_199091189__/RConn3 -- bus587/LConn1
  T_46971910__/RConn1 -- L_46971910/LConn1
  T_46971910__/RConn2 -- L_46971910/LConn2
  L_46971910/LConn3 -- T_46971910__/RConn3 -- bus588/LConn1
  T_198351119__/RConn1 -- L_198351119/LConn1
  T_198351119__/RConn2 -- L_198351119/LConn2
  L_198351119/LConn3 -- T_198351119__/RConn3 -- bus589/LConn1
  T_198331310__/RConn1 -- L_198331310/LConn1
  T_198331310__/RConn2 -- L_198331310/LConn2
  L_198331310/LConn3 -- T_198331310__/RConn3 -- bus590/LConn1
  T_198330048__/RConn1 -- L_198330048/LConn1
  T_198330048__/RConn2 -- L_198330048/LConn2
  L_198330048/LConn3 -- T_198330048__/RConn3 -- bus591/LConn1
  T_132976488__Berri_Gas_Plant/RConn1 -- L_132976488/LConn1
  T_132976488__Berri_Gas_Plant/RConn2 -- L_132976488/LConn2
  L_132976488/LConn3 -- T_132976488__Berri_Gas_Plant/RConn3 -- bus592/LConn1
  T_198342216__/RConn1 -- L_198342216/LConn1
  T_198342216__/RConn2 -- L_198342216/LConn2
  L_198342216/LConn3 -- T_198342216__/RConn3 -- bus593/LConn1
  T_168652821__/RConn1 -- L_168652821/LConn1
  T_168652821__/RConn2 -- L_168652821/LConn2
  L_168652821/LConn3 -- T_168652821__/RConn3 -- bus594/LConn1
  T_198358326__/RConn1 -- L_198358326/LConn1
  T_198358326__/RConn2 -- L_198358326/LConn2
  L_198358326/LConn3 -- T_198358326__/RConn3 -- bus595/LConn1
  T_188546296__/RConn1 -- L_188546296/LConn1
  T_188546296__/RConn2 -- L_188546296/LConn2
  L_188546296/LConn3 -- T_188546296__/RConn3 -- bus596/LConn1
  T_198334634__/RConn1 -- L_198334634/LConn1
  T_198334634__/RConn2 -- L_198334634/LConn2
  L_198334634/LConn3 -- T_198334634__/RConn3 -- bus597/LConn1
  T_198144511__/RConn1 -- L_198144511/LConn1
  T_198144511__/RConn2 -- L_198144511/LConn2
  L_198144511/LConn3 -- T_198144511__/RConn3 -- bus598/LConn1
  T_195637944__/RConn1 -- L_195637944/LConn1
  T_195637944__/RConn2 -- L_195637944/LConn2
  L_195637944/LConn3 -- T_195637944__/RConn3 -- bus599/LConn1
  T_197445313__/RConn1 -- L_197445313/LConn1
  T_197445313__/RConn2 -- L_197445313/LConn2
  L_197445313/LConn3 -- T_197445313__/RConn3 -- bus600/LConn1
  T_168648926__/RConn1 -- L_168648926/LConn1
  T_168648926__/RConn2 -- L_168648926/LConn2
  L_168648926/LConn3 -- T_168648926__/RConn3 -- bus601/LConn1
  T_115326819__/RConn1 -- L_115326819/LConn1
  T_115326819__/RConn2 -- L_115326819/LConn2
  L_115326819/LConn3 -- T_115326819__/RConn3 -- bus602/LConn1
  T_197662314__/RConn1 -- L_197662314/LConn1
  T_197662314__/RConn2 -- L_197662314/LConn2
  L_197662314/LConn3 -- T_197662314__/RConn3 -- bus603/LConn1
  T_197432428__/RConn1 -- L_197432428/LConn1
  T_197432428__/RConn2 -- L_197432428/LConn2
  L_197432428/LConn3 -- T_197432428__/RConn3 -- bus604/LConn1
  T_197442799__/RConn1 -- L_197442799/LConn1
  T_197442799__/RConn2 -- L_197442799/LConn2
  L_197442799/LConn3 -- T_197442799__/RConn3 -- bus605/LConn1
  T_197439486__/RConn1 -- L_197439486/LConn1
  T_197439486__/RConn2 -- L_197439486/LConn2
  L_197439486/LConn3 -- T_197439486__/RConn3 -- bus606/LConn1
  T_261938325__/RConn1 -- L_261938325/LConn1
  T_261938325__/RConn2 -- L_261938325/LConn2
  L_261938325/LConn3 -- T_261938325__/RConn3 -- bus607/LConn1
  T_160398714__/RConn1 -- L_160398714/LConn1
  T_160398714__/RConn2 -- L_160398714/LConn2
  L_160398714/LConn3 -- T_160398714__/RConn3 -- bus608/LConn1
  T_203618603__/RConn1 -- L_203618603/LConn1
  T_203618603__/RConn2 -- L_203618603/LConn2
  L_203618603/LConn3 -- T_203618603__/RConn3 -- bus609/LConn1
  T_132154027__/RConn1 -- L_132154027/LConn1
  T_132154027__/RConn2 -- L_132154027/LConn2
  L_132154027/LConn3 -- T_132154027__/RConn3 -- bus610/LConn1
  T_203622084__/RConn1 -- L_203622084/LConn1
  T_203622084__/RConn2 -- L_203622084/LConn2
  L_203622084/LConn3 -- T_203622084__/RConn3 -- bus611/LConn1
  T_203622086__/RConn1 -- L_203622086/LConn1
  T_203622086__/RConn2 -- L_203622086/LConn2
  L_203622086/LConn3 -- T_203622086__/RConn3 -- bus612/LConn1
  T_203622279__/RConn1 -- L_203622279/LConn1
  T_203622279__/RConn2 -- L_203622279/LConn2
  L_203622279/LConn3 -- T_203622279__/RConn3 -- bus613/LConn1
  "T_261938316__Substation_Al_Omariya_\"W\""/RConn1 -- L_261938316/LConn1
  "T_261938316__Substation_Al_Omariya_\"W\""/RConn2 -- L_261938316/LConn2
  L_261938316/LConn3 -- "T_261938316__Substation_Al_Omariya_\"W\""/RConn3 -- bus614/LConn1
  T_203855651__/RConn1 -- L_203855651/LConn1
  T_203855651__/RConn2 -- L_203855651/LConn2
  L_203855651/LConn3 -- T_203855651__/RConn3 -- bus615/LConn1
  T_132154028__Substation/RConn1 -- L_132154028/LConn1
  T_132154028__Substation/RConn2 -- L_132154028/LConn2
  L_132154028/LConn3 -- T_132154028__Substation/RConn3 -- bus616/LConn1
  T_203858094__/RConn1 -- L_203858094/LConn1
  T_203858094__/RConn2 -- L_203858094/LConn2
  L_203858094/LConn3 -- T_203858094__/RConn3 -- bus617/LConn1
  T_203618746__/RConn1 -- L_203618746/LConn1
  T_203618746__/RConn2 -- L_203618746/LConn2
  L_203618746/LConn3 -- T_203618746__/RConn3 -- bus618/LConn1
  T_196903043__/RConn1 -- L_196903043/LConn1
  T_196903043__/RConn2 -- L_196903043/LConn2
  L_196903043/LConn3 -- T_196903043__/RConn3 -- bus619/LConn1
  T_115345577__/RConn1 -- L_115345577/LConn1
  T_115345577__/RConn2 -- L_115345577/LConn2
  L_115345577/LConn3 -- T_115345577__/RConn3 -- bus620/LConn1
  T_196917881__/RConn1 -- L_196917881/LConn1
  T_196917881__/RConn2 -- L_196917881/LConn2
  L_196917881/LConn3 -- T_196917881__/RConn3 -- bus621/LConn1
  T_187924742__/RConn1 -- L_187924742/LConn1
  T_187924742__/RConn2 -- L_187924742/LConn2
  L_187924742/LConn3 -- T_187924742__/RConn3 -- bus622/LConn1
  T_331253129__/RConn1 -- L_331253129/LConn1
  T_331253129__/RConn2 -- L_331253129/LConn2
  L_331253129/LConn3 -- T_331253129__/RConn3 -- bus623/LConn1
  T_115345561__/RConn1 -- L_115345561/LConn1
  T_115345561__/RConn2 -- L_115345561/LConn2
  L_115345561/LConn3 -- T_115345561__/RConn3 -- bus624/LConn1
  T_168652806__/RConn1 -- L_168652806/LConn1
  T_168652806__/RConn2 -- L_168652806/LConn2
  L_168652806/LConn3 -- T_168652806__/RConn3 -- bus625/LConn1
  T_115345550__/RConn1 -- L_115345550/LConn1
  T_115345550__/RConn2 -- L_115345550/LConn2
  L_115345550/LConn3 -- T_115345550__/RConn3 -- bus626/LConn1
  T_115345535__/RConn1 -- L_115345535/LConn1
  T_115345535__/RConn2 -- L_115345535/LConn2
  L_115345535/LConn3 -- T_115345535__/RConn3 -- bus627/LConn1
  T_190221971__/RConn1 -- L_190221971/LConn1
  T_190221971__/RConn2 -- L_190221971/LConn2
  L_190221971/LConn3 -- T_190221971__/RConn3 -- bus628/LConn1
  T_195636040__/RConn1 -- L_195636040/LConn1
  T_195636040__/RConn2 -- L_195636040/LConn2
  L_195636040/LConn3 -- T_195636040__/RConn3 -- bus629/LConn1
  T_204824991__/RConn1 -- L_204824991/LConn1
  T_204824991__/RConn2 -- L_204824991/LConn2
  L_204824991/LConn3 -- T_204824991__/RConn3 -- bus630/LConn1
  T_194977916__/RConn1 -- L_194977916/LConn1
  T_194977916__/RConn2 -- L_194977916/LConn2
  L_194977916/LConn3 -- T_194977916__/RConn3 -- bus631/LConn1
  T_115345572__/RConn1 -- L_115345572/LConn1
  T_115345572__/RConn2 -- L_115345572/LConn2
  L_115345572/LConn3 -- T_115345572__/RConn3 -- bus632/LConn1
  T_115345575__/RConn1 -- L_115345575/LConn1
  T_115345575__/RConn2 -- L_115345575/LConn2
  L_115345575/LConn3 -- T_115345575__/RConn3 -- bus633/LConn1
  T_115204773__/RConn1 -- L_115204773/LConn1
  T_115204773__/RConn2 -- L_115204773/LConn2
  L_115204773/LConn3 -- T_115204773__/RConn3 -- bus634/LConn1
  T_203627872__/RConn1 -- L_203627872/LConn1
  T_203627872__/RConn2 -- L_203627872/LConn2
  L_203627872/LConn3 -- T_203627872__/RConn3 -- bus635/LConn1
  T_197252542__/RConn1 -- L_197252542/LConn1
  T_197252542__/RConn2 -- L_197252542/LConn2
  L_197252542/LConn3 -- T_197252542__/RConn3 -- bus636/LConn1
  T_115188425__/RConn1 -- L_115188425/LConn1
  T_115188425__/RConn2 -- L_115188425/LConn2
  L_115188425/LConn3 -- T_115188425__/RConn3 -- bus637/LConn1
  T_115168488__/RConn1 -- L_115168488/LConn1
  T_115168488__/RConn2 -- L_115168488/LConn2
  L_115168488/LConn3 -- T_115168488__/RConn3 -- bus638/LConn1
  T_52609387__/RConn1 -- L_52609387/LConn1
  T_52609387__/RConn2 -- L_52609387/LConn2
  L_52609387/LConn3 -- T_52609387__/RConn3 -- bus639/LConn1
  T_45103712__/RConn1 -- L_45103712/LConn1
  T_45103712__/RConn2 -- L_45103712/LConn2
  L_45103712/LConn3 -- T_45103712__/RConn3 -- bus640/LConn1
  T_205485383__/RConn1 -- L_205485383/LConn1
  T_205485383__/RConn2 -- L_205485383/LConn2
  L_205485383/LConn3 -- T_205485383__/RConn3 -- bus641/LConn1
  T_205485574__/RConn1 -- L_205485574/LConn1
  T_205485574__/RConn2 -- L_205485574/LConn2
  L_205485574/LConn3 -- T_205485574__/RConn3 -- bus642/LConn1
  T_204787949__/RConn1 -- L_204787949/LConn1
  T_204787949__/RConn2 -- L_204787949/LConn2
  L_204787949/LConn3 -- T_204787949__/RConn3 -- bus643/LConn1
  T_115326806_380000_/RConn1 -- L_115326806/LConn1
  T_115326806_380000_/RConn2 -- L_115326806/LConn2
  L_115326806/LConn3 -- T_115326806_380000_/RConn3 -- bus644/LConn1
  T_207785816__/RConn1 -- L_207785816/LConn1
  T_207785816__/RConn2 -- L_207785816/LConn2
  L_207785816/LConn3 -- T_207785816__/RConn3 -- bus645/LConn1
  T_196291944__/RConn1 -- L_196291944/LConn1
  T_196291944__/RConn2 -- L_196291944/LConn2
  L_196291944/LConn3 -- T_196291944__/RConn3 -- bus646/LConn1
  T_195156716__/RConn1 -- L_195156716/LConn1
  T_195156716__/RConn2 -- L_195156716/LConn2
  L_195156716/LConn3 -- T_195156716__/RConn3 -- bus647/LConn1
  T_209263045__/RConn1 -- L_209263045/LConn1
  T_209263045__/RConn2 -- L_209263045/LConn2
  L_209263045/LConn3 -- T_209263045__/RConn3 -- bus648/LConn1
  T_216869978__/RConn1 -- L_216869978/LConn1
  T_216869978__/RConn2 -- L_216869978/LConn2
  L_216869978/LConn3 -- T_216869978__/RConn3 -- bus649/LConn1
  T_231599971__/RConn1 -- L_231599971/LConn1
  T_231599971__/RConn2 -- L_231599971/LConn2
  L_231599971/LConn3 -- T_231599971__/RConn3 -- bus650/LConn1
  T_194977895__/RConn1 -- L_194977895/LConn1
  T_194977895__/RConn2 -- L_194977895/LConn2
  L_194977895/LConn3 -- T_194977895__/RConn3 -- bus651/LConn1
  T_197434236__/RConn1 -- L_197434236/LConn1
  T_197434236__/RConn2 -- L_197434236/LConn2
  L_197434236/LConn3 -- T_197434236__/RConn3 -- bus652/LConn1
  T_309146009__Sila/RConn1 -- L_309146009/LConn1
  T_309146009__Sila/RConn2 -- L_309146009/LConn2
  L_309146009/LConn3 -- T_309146009__Sila/RConn3 -- bus653/LConn1
  T_186499524__Salwa/RConn1 -- L_186499524/LConn1
  T_186499524__Salwa/RConn2 -- L_186499524/LConn2
  L_186499524/LConn3 -- T_186499524__Salwa/RConn3 -- bus654/LConn1
  T_385901993__/RConn1 -- L_385901993/LConn1
  T_385901993__/RConn2 -- L_385901993/LConn2
  L_385901993/LConn3 -- T_385901993__/RConn3 -- bus655/LConn1
  T_375827318__/RConn1 -- L_375827318/LConn1
  T_375827318__/RConn2 -- L_375827318/LConn2
  L_375827318/LConn3 -- T_375827318__/RConn3 -- bus656/LConn1
  T_29495366__/RConn1 -- L_29495366/LConn1
  T_29495366__/RConn2 -- L_29495366/LConn2
  L_29495366/LConn3 -- T_29495366__/RConn3 -- bus657/LConn1
  T_29497443__/RConn1 -- L_29497443/LConn1
  T_29497443__/RConn2 -- L_29497443/LConn2
  L_29497443/LConn3 -- T_29497443__/RConn3 -- bus658/LConn1
  T_173064710__/RConn1 -- L_173064710/LConn1
  T_173064710__/RConn2 -- L_173064710/LConn2
  L_173064710/LConn3 -- T_173064710__/RConn3 -- bus659/LConn1
  T_29497493__/RConn1 -- L_29497493/LConn1
  T_29497493__/RConn2 -- L_29497493/LConn2
  L_29497493/LConn3 -- T_29497493__/RConn3 -- bus660/LConn1
  T_94816872__/RConn1 -- L_94816872/LConn1
  T_94816872__/RConn2 -- L_94816872/LConn2
  L_94816872/LConn3 -- T_94816872__/RConn3 -- bus661/LConn1
  T_359425700__Barsha/RConn1 -- L_359425700/LConn1
  T_359425700__Barsha/RConn2 -- L_359425700/LConn2
  L_359425700/LConn3 -- T_359425700__Barsha/RConn3 -- bus662/LConn1
  T_24510596__/RConn1 -- L_24510596/LConn1
  T_24510596__/RConn2 -- L_24510596/LConn2
  L_24510596/LConn3 -- T_24510596__/RConn3 -- bus663/LConn1
  T_181332757__DEWA/RConn1 -- L_181332757/LConn1
  T_181332757__DEWA/RConn2 -- L_181332757/LConn2
  L_181332757/LConn3 -- T_181332757__DEWA/RConn3 -- bus664/LConn1
  T_181332762__/RConn1 -- L_181332762/LConn1
  T_181332762__/RConn2 -- L_181332762/LConn2
  L_181332762/LConn3 -- T_181332762__/RConn3 -- bus665/LConn1
  T_173064712__/RConn1 -- L_173064712/LConn1
  T_173064712__/RConn2 -- L_173064712/LConn2
  L_173064712/LConn3 -- T_173064712__/RConn3 -- bus666/LConn1
  T_149865727__/RConn1 -- L_149865727/LConn1
  T_149865727__/RConn2 -- L_149865727/LConn2
  L_149865727/LConn3 -- T_149865727__/RConn3 -- bus667/LConn1
  T_94950821__/RConn1 -- L_94950821/LConn1
  T_94950821__/RConn2 -- L_94950821/LConn2
  L_94950821/LConn3 -- T_94950821__/RConn3 -- bus668/LConn1
  T_198117361__Al_Fadhili_back_to_back_HVDC_converter_station/RConn1 -- L_198117361/LConn1
  T_198117361__Al_Fadhili_back_to_back_HVDC_converter_station/RConn2 -- L_198117361/LConn2
  L_198117361/LConn3 -- T_198117361__Al_Fadhili_back_to_back_HVDC_converter_station/RConn3 -- bus669/LConn1
  T_174871442__/RConn1 -- L_174871442/LConn1
  T_174871442__/RConn2 -- L_174871442/LConn2
  L_174871442/LConn3 -- T_174871442__/RConn3 -- bus670/LConn1
  T_94816851__/RConn1 -- L_94816851/LConn1
  T_94816851__/RConn2 -- L_94816851/LConn2
  L_94816851/LConn3 -- T_94816851__/RConn3 -- bus671/LConn1
  T_354339381__/RConn1 -- L_354339381/LConn1
  T_354339381__/RConn2 -- L_354339381/LConn2
  L_354339381/LConn3 -- T_354339381__/RConn3 -- bus672/LConn1
  T_94950807__/RConn1 -- L_94950807/LConn1
  T_94950807__/RConn2 -- L_94950807/LConn2
  L_94950807/LConn3 -- T_94950807__/RConn3 -- bus673/LConn1
  T_196917879__/RConn1 -- L_196917879/LConn1
  T_196917879__/RConn2 -- L_196917879/LConn2
  L_196917879/LConn3 -- T_196917879__/RConn3 -- bus674/LConn1
  T_186404765__/RConn1 -- L_186404765/LConn1
  T_186404765__/RConn2 -- L_186404765/LConn2
  L_186404765/LConn3 -- T_186404765__/RConn3 -- bus675/LConn1
  T_186404770_400000_/RConn1 -- L_186404770/LConn1
  T_186404770_400000_/RConn2 -- L_186404770/LConn2
  L_186404770/LConn3 -- T_186404770_400000_/RConn3 -- bus676/LConn1
  T_177998754__/RConn1 -- L_177998754/LConn1
  T_177998754__/RConn2 -- L_177998754/LConn2
  L_177998754/LConn3 -- T_177998754__/RConn3 -- bus677/LConn1
  T_321061210__/RConn1 -- L_321061210/LConn1
  T_321061210__/RConn2 -- L_321061210/LConn2
  L_321061210/LConn3 -- T_321061210__/RConn3 -- bus678/LConn1
  T_260963602__/RConn1 -- L_260963602/LConn1
  T_260963602__/RConn2 -- L_260963602/LConn2
  L_260963602/LConn3 -- T_260963602__/RConn3 -- bus679/LConn1
  T_169873584__/RConn1 -- L_169873584/LConn1
  T_169873584__/RConn2 -- L_169873584/LConn2
  L_169873584/LConn3 -- T_169873584__/RConn3 -- bus680/LConn1
  T_186488516__Um_Birka_Super/RConn1 -- L_186488516/LConn1
  T_186488516__Um_Birka_Super/RConn2 -- L_186488516/LConn2
  L_186488516/LConn3 -- T_186488516__Um_Birka_Super/RConn3 -- bus681/LConn1
  T_186488517__/RConn1 -- L_186488517/LConn1
  T_186488517__/RConn2 -- L_186488517/LConn2
  L_186488517/LConn3 -- T_186488517__/RConn3 -- bus682/LConn1
  T_29494113__/RConn1 -- L_29494113/LConn1
  T_29494113__/RConn2 -- L_29494113/LConn2
  L_29494113/LConn3 -- T_29494113__/RConn3 -- bus683/LConn1
  T_375782393__/RConn1 -- L_375782393/LConn1
  T_375782393__/RConn2 -- L_375782393/LConn2
  L_375782393/LConn3 -- T_375782393__/RConn3 -- bus684/LConn1
  T_375782394__/RConn1 -- L_375782394/LConn1
  T_375782394__/RConn2 -- L_375782394/LConn2
  L_375782394/LConn3 -- T_375782394__/RConn3 -- bus685/LConn1
